simulink model "mc_pos"  (R2021a)
settings: Solver=FixedStepAuto  StartTime=0.0  StopTime=10.0  FixedStep=0.1  RelTol=1e-3
undefined symbols (not defined in the file): CONSTANTS_ONE_G, DiscIntNeverNeededParam, MPC_LAND_SPEED, MPC_SPOOLUP_TIME, MPC_THR_HOVER, MPC_THR_MAX, MPC_THR_MIN, MPC_TILTMAX_AIR, MPC_TILTMAX_LND, MPC_TKO_RAMP_T, MPC_VELD_LP, MPC_XY_P, MPC_XY_VEL_D_ACC, MPC_XY_VEL_I_ACC, MPC_XY_VEL_MAX, MPC_XY_VEL_P_ACC, MPC_Z_P, MPC_Z_VEL_D_ACC, MPC_Z_VEL_I_ACC, MPC_Z_VEL_MAX_DN, MPC_Z_VEL_MAX_UP, MPC_Z_VEL_P_ACC, PX4_TAKEOFF_STATUS, WV_EN
libraries: simulink x16, vrlib x2, sharedtransform x2, aerolibconvert2 x1
(part 3 of 3)

== stateflow chart mc_pos/Flight Mode Manager/Flight Task ==
  state switch_flight_task [parallel]
    en,du:
    start_flight_task();
    handleCommand();
    settings: executionOrder=1
    state Switch_Flight_Task
      state VTOL
        state VTOL_FW_Mode
          en:
          sprintf("Do not run any flight task for VTOLs in fixed-wing mode")
          du:
        state TRANSITION
          en,du:
          task_ == PX4_FLIGHT_TASK.TRANSITION;
        (junction 861) -> VTOL_FW_Mode [order 1] : [vehicle_status.vehicle_type == ...
            | PX4_VEHICLE_STATUS.VEHICLE_TYPE_FIXED_WING]
        (junction 861) -> (junction 859) [order 2]
        (junction 859) -> TRANSITION [order 1] : [vehicle_status.in_transition_mode && ...
            | control_mode.flag_control_altitude_enabled]
      state AUTO
        state AUTO_FOLLOW_ME
          en,du:
          task_ == PX4_FLIGHT_TASK.AUTO_FOLLOW_ME;
        state DESCEND
          en,du:
          task_ == PX4_FLIGHT_TASK.DESCEND;
        state AUTO_LINE_SMOOTH_VEL
          en,du:
          task_ == PX4_FLIGHT_TASK.AUTO_LINE_SMOOTH_VEL;
        (junction 863) -> AUTO_FOLLOW_ME [order 1] : [vehicle_status.nav_state == ...
            | PX4_VEHICLE_STATUS.NAVIGATION_STATE_AUTO_FOLLOW_TARGET]
        (junction 867) -> DESCEND [order 1] : [vehicle_status.nav_state == ...
            | PX4_VEHICLE_STATUS.NAVIGATION_STATE_DESCEND]
        (junction 863) -> (junction 865) [order 2]
        (junction 865) -> (junction 867) [order 2]
        (junction 865) -> AUTO_LINE_SMOOTH_VEL [order 1] : [control_mode.flag_control_auto_enabled]
      state MANUAL
        state MANUAL_POSITION_SMOOTH_VEL
          en,du:
          task_ == PX4_FLIGHT_TASK.MANUAL_POSITION_SMOOTH_VEL;
        state MANUAL_ALTITUDE
          en,du:
          task_ == PX4_FLIGHT_TASK.MANUAL_ALTITUDE;
        state MANUAL_POSITION
          en,du:
          task_ == PX4_FLIGHT_TASK.MANUAL_POSITION;
        state MANUAL_ACCELERATION
          en,du:
          task_ == PX4_FLIGHT_TASK.MANUAL_ACCELERATION;
        state MANUAL_ALTITUDE_SMOOTH_VEL
          en,du:
          task_ == PX4_FLIGHT_TASK.MANUAL_ALTITUDE_SMOOTH_VEL;
        (junction 888) -> MANUAL_POSITION_SMOOTH_VEL [order 1] : [vehicle_status.nav_state == ...
            | PX4_VEHICLE_STATUS.NAVIGATION_STATE_ALTCTL && ...
            | MPC_POS_MODE == 3]
        (junction 872) -> MANUAL_ALTITUDE [order 1] : [vehicle_status.nav_state == ...
            | PX4_VEHICLE_STATUS.NAVIGATION_STATE_ALTCTL && ...
            | MPC_POS_MODE == 0]
        (junction 876) -> (junction 888) [order 2]
        (junction 888) -> (junction 874) [order 2]
        (junction 874) -> (junction 872) [order 2]
        (junction 872) -> (junction 803) [order 2]
        (junction 876) -> MANUAL_POSITION [order 1] : [vehicle_status.nav_state == ...
            | PX4_VEHICLE_STATUS.NAVIGATION_STATE_POSCTL && ...
            | MPC_POS_MODE == 0]
        (junction 874) -> MANUAL_ACCELERATION [order 1] : [vehicle_status.nav_state == ...
            | PX4_VEHICLE_STATUS.NAVIGATION_STATE_POSCTL]
        (junction 803) -> MANUAL_ALTITUDE_SMOOTH_VEL [order 1] : [vehicle_status.nav_state == ....
            | PX4_VEHICLE_STATUS.NAVIGATION_STATE_POSCTL && ...
            | MPC_POS_MODE == 3]
      state OTHER
        state NAVIGATION_STATE_ORBIT
        state None
        (junction 899) -> NAVIGATION_STATE_ORBIT [order 1] : [vehicle_status.nav_state == ...
            | PX4_VEHICLE_STATUS.NAVIGATION_STATE_ORBIT]
        (junction 899) -> None [order 2]
      (default) -> (junction 797)
      (junction 797) -> (junction 861)
      (junction 859) -> (junction 863) [order 2]
      (junction 867) -> (junction 876) [order 2]
      Switch_Flight_Task -> (junction 797) : [hasChanged(local_position.timestamp)]
      (junction 803) -> (junction 899) [order 2]
  state mode_action [parallel]
    settings: executionOrder=2
    state Transition [parallel]
      settings: executionOrder=1
      state running
        en,du:
        % update_initial阶段, 初始化时间和输入数据
        mode_action.FlightTask_updateInitialize();
        % update垂起的过渡阶段，将垂直速度和水平姿态的setpoint点置0
        checkEkfResetCounters();
        acceleration_setpoint(1) = single(0.0);
        acceleration_setpoint(2) = single(0.0);
        position_setpoint = [single(nan); single(nan); single(nan)];
        velocity_setpoint(3) = single(0.0);
        yaw_setpoint = single(nan);
        % update_finalize阶段：在update()之后调用
        %来约束生成的设定值，以符合当前模式的约束
        % update_finalize_none
        takeoff_reactivate
      state not_run
      (default) -> mode_action.Transition.not_run
      mode_action.Transition.not_run -> mode_action.Transition.running : [task_ == PX4_FLIGHT_TASK.TRANSITION]
      mode_action.Transition.running -> mode_action.Transition.not_run : [task_ ~= PX4_FLIGHT_TASK.TRANSITION]
    state AutoFollowMe [parallel]
      settings: executionOrder=2
    state AutoLineSmoothVel [parallel]
      settings: executionOrder=10
      state running
        en,du:
        ext_yaw_handler = weather_vane;
        FlightTaskAuto_updateInitialize
        FlightTaskAutoMapper_update
        FlightTaskAuto_updateFinalize
        takeoff_reactivate
      state not_run
      (default) -> mode_action.AutoLineSmoothVel.not_run
      mode_action.AutoLineSmoothVel.not_run -> mode_action.AutoLineSmoothVel.running : [task_ == PX4_FLIGHT_TASK.AUTO_LINE_SMOOTH_VEL]
      mode_action.AutoLineSmoothVel.running -> mode_action.AutoLineSmoothVel.not_run : [task_ ~= PX4_FLIGHT_TASK.AUTO_LINE_SMOOTH_VEL]
    state Descend [parallel]
      settings: executionOrder=3
    state ManualPosition [parallel]
      settings: executionOrder=4
      state running
        en,du:
        weathervane_yaw_handler = weather_vane;
        % update_initial
        FlightTask_updateInitialize
        Sticks_checkAndSetStickInputs
        % update
        ManualPosition_checkEkfResetCounters
        FlightTaskManualAltitude_updateConstraintsFromEstimator
        ManualPosition_scaleSticks
        ManualPosition_updateSetpoints
        constraints.want_takeoff = (stick_positions_(3) < -0.3);
        % update_final_none
        takeoff_reactivate
      state not_run
      (default) -> mode_action.ManualPosition.not_run
      mode_action.ManualPosition.not_run -> mode_action.ManualPosition.running : [task_==PX4_FLIGHT_TASK.MANUAL_POSITION]
      mode_action.ManualPosition.running -> mode_action.ManualPosition.not_run : [task_~=PX4_FLIGHT_TASK.MANUAL_POSITION]
    state ManualPositionSmoothVel_checking [parallel]
      settings: executionOrder=5
      state not_run
      state running
        en,du:
        weathervane_yaw_handler = weather_vane;
        % update_initial
        mode_action.FlightTask_updateInitialize();
        mode_action.Sticks_checkAndSetStickInputs();
        % update
        ManualPositionSmoothVel_checkEkfResetCounters();
        FlightTaskManualAltitude_updateConstraintsFromEstimator();
        ManualPositionSmoothVel_scaleSticks();
        ManualPositionSmoothVel_updateSetpoints();
        constraints.want_takeoff = (stick_positions_(3) < -0.3);
        % update_finalize_none
        takeoff_reactivate();
      (default) -> mode_action.ManualPositionSmoothVel_checking.not_run
      mode_action.ManualPositionSmoothVel_checking.not_run -> mode_action.ManualPositionSmoothVel_checking.running : [(task_ == PX4_FLIGHT_TASK.MANUAL_POSITION_SMOOTH_VEL)  && ...
          |  (switchTask() == PX4_FLIGHT_TASK_ERROR.NO_ERROR)]
      mode_action.ManualPositionSmoothVel_checking.running -> mode_action.ManualPositionSmoothVel_checking.not_run : [task_ ~= PX4_FLIGHT_TASK.MANUAL_POSITION_SMOOTH_VEL]
    state ManualAcceleration [parallel]
      settings: executionOrder=6
    state ManualAltitude [parallel]
      settings: executionOrder=7
      state running
        en,du:
        % update_initial
        FlightTask_updateInitialize
        Sticks_checkAndSetStickInputs
        % update
        ManualAltitude_checkEkfResetCounters
        FlightTaskManualAltitude_updateConstraintsFromEstimator
        ManualAltitude_scaleSticks
        ManualAltitude_updateSetpoints
        constraints.want_takeoff = (stick_positions_(3) < -0.3);
        % update_finalize_none
        takeoff_reactivate
      state not_run
      (default) -> mode_action.ManualAltitude.not_run
      mode_action.ManualAltitude.not_run -> mode_action.ManualAltitude.running : [task_ == PX4_FLIGHT_TASK.MANUAL_ALTITUDE]
      mode_action.ManualAltitude.running -> mode_action.ManualAltitude.not_run : [task_ ~= PX4_FLIGHT_TASK.MANUAL_ALTITUDE]
    state ManualAltitudeSmoothVel [parallel]
      settings: executionOrder=8
      state running
        en,du:
        % update_initial
        FlightTask_updateInitialize();
        Sticks_checkAndSetStickInputs();
        % update
        ManualAltitudeSmoothVel_checkEkfResetCounters();
        FlightTaskManualAltitude_updateConstraintsFromEstimator();
        ManualAltitudeSmoothVel_scaleSticks();
        ManualAltitudeSmoothVel_updateSetpoints();
        constraints.want_takeoff = (stick_positions_(3) < -0.3);
        % update_finalize_none
        takeoff_reactivate();
      state not_run
      (default) -> mode_action.ManualAltitudeSmoothVel.not_run
      mode_action.ManualAltitudeSmoothVel.not_run -> mode_action.ManualAltitudeSmoothVel.running : [task_==PX4_FLIGHT_TASK.MANUAL_ALTITUDE_SMOOTH_VEL]
      mode_action.ManualAltitudeSmoothVel.running -> mode_action.ManualAltitudeSmoothVel.not_run : [task_~=PX4_FLIGHT_TASK.MANUAL_ALTITUDE_SMOOTH_VEL]
    state Failsafe [parallel]
      settings: executionOrder=9
      state running
        en,du:
        % update initial
        FlightTask_updateInitialize
        % update
        Failsafe_update
        % update_finalize_none
        takeoff_reactivate
      state not_run
      (default) -> mode_action.Failsafe.not_run
      mode_action.Failsafe.not_run -> mode_action.Failsafe.running : [task_ == PX4_FLIGHT_TASK.FAILSAFE]
      mode_action.Failsafe.running -> mode_action.Failsafe.not_run : [task_ ~= PX4_FLIGHT_TASK.FAILSAFE]
  data: out function_output; out function_output; out function_output; out function_output; type local uint8; target_acceptance_radius local single size=1; target local single size=3 =[single(nan); single(nan); single(nan)]; prev_wp local single size=3 =[single(nan); single(nan); single(nan)]; next_wp local single size=3 =[single(nan); single(nan); single(nan)]; mc_cruise_speed local single size=1; reference_position local Bus: px4_reference_position; reference_altitude local single size=1; current_state local Enum: PX4_FLIGHT_TASK_INTERNAL_STATE size=1; closest_pt local single size=2 =[single(nan); single(nan)]; yaw_lock local boolean size=1; wantTakeoff local boolean =false; yaw_sp_aligned local boolean =false; yaw_sp_prev local single size=1 =single(nan); ext_yaw_handler local Bus: px4_weather_vane; trajectory local Bus: px4_mc_pos_traj size=3; out function_output; velocity_scale local single size=1; weathervane_yaw_handler local Bus: px4_weather_vane; result function_output; position_estimate local single size=3; position_lock_active_xy local boolean size=1; position_lock_active_z local boolean size=1; position_setpoint_locked local single size=3; velocity_scale local single size=1; weathervane_yaw_handler local Bus: px4_weather_vane; trajectory local Bus: px4_mc_pos_traj size=3; result function_output; out function_output; position_lock_active_z local boolean size=1; position_setpoint_locked local single size=1; position_estimate local single size=1; trajectory local Bus: px4_mc_pos_traj size=1; out function_output; input_available function_output; dt function_input; time_stretch function_input; traj function_input; out function_output; vel_setpoint function_input; traj function_input; out function_output; traj function_input; n_traj function_input; out function_output; u function_input; out function_output; apply_brake function_input; stopped function_input; d_to_g_lock function_input; out function_output; dcm_z function_input; yyaw function_input; out function_output; weather_vane input Bus: px4_weather_vane size=1; position_setpoint_input input Bus: px4_vehicle_local_position_setpoint; control_mode input Bus: px4_vehicle_control_mode; constraints output Bus: px4_vehicle_constraints; position_ local single size=3; velocity_ local single size=3; yaw_ local single size=1; MPC_XY_CRUISE parameter single; MPC_ACC_HOR parameter single; MPC_JERK_AUTO parameter single; MPC_ACC_DOWN_MAX parameter single; MPC_Z_VEL_MAX_DN parameter single; MPC_XY_VEL_MAX parameter single; dist_to_bottom_ local single size=1; local_position input Bus: px4_vehicle_local_position; home_position input Bus: px4_home_position; dist_to_ground_ local single size=1; triplet_setpoint input Bus: px4_position_setpoint_triplet; MPC_Z_VEL_MAX_UP parameter single; CONSTANTS_RADIUS_OF_EARTH parameter double; MPC_YAW_MODE parameter int32; MPC_ACC_UP_MAX parameter single; MPC_LAND_ALT1 parameter single; MPC_TKO_SPEED parameter single; MPC_TKO_RAMP_T parameter single; manual_control_setpoint input Bus: px4_manual_control_setpoint; positions_expo_ local single size=4 =single([0.0; 0.0; 0.0; 0.0]); vehicle_status input Bus: px4_vehicle_status; MPC_LAND_ALT2 parameter single; MPC_LAND_SPEED parameter single; MPC_LAND_RC_HELP parameter int32; MPC_XY_MAN_EXPO parameter single; MPC_Z_MAN_EXPO parameter single; MPC_YAW_EXPO parameter single; MPC_HOLD_DZ parameter single; NAV_MC_ALT_RAD parameter single; MPC_XY_TRAJ_P parameter single; MPC_XY_ERR_MAX parameter single; deltatime_ local size=1; MPC_YAWRAUTO_MAX parameter single; MIS_YAW_ERR parameter single; MPC_VEL_MANUAL parameter single; stick_positions_ local single size=4 =single([0.0; 0.0; 0.0; 0.0]); MPC_MAN_Y_MAX parameter single; MPC_MAN_Y_TAU parameter single; MPC_JERK_MAX parameter single; MPC_ACC_HOR_MAX parameter single; velocity_setpoint_feedback_ local single size=3; MC_MAN_TILT_TAU parameter single; MPC_MAN_TILT_MAX parameter single; MPC_HOLD_MAX_Z parameter single; MPC_ALT_MODE parameter int32; MPC_HOLD_MAX_XY parameter single; MPC_Z_P parameter single; max_distance_to_ground_ local single size=1; min_distance_to_ground_ local single size=1; max_speed_up_ local single size=1; max_speed_down_ local single size=1; CONSTANTS_ONE_G parameter single size=1; reset_counter_xy_ local uint8 size=1 =uint8(0); reset_counter_vxy_ local uint8 size=1 =uint8(0); reset_counter_z_ local uint8 size=1 =uint8(0); reset_counter_vz_ local uint8 size=1 =uint8(0); reset_counter_heading_ local uint8 size=1 =uint8(0); time_stamp_last_ local size=1 =0; WV_ROLL_MIN parameter single size=1; WV_GAIN parameter single size=1; WV_YRATE_MAX parameter single size=1; WV_EN parameter boolean size=1; task_ local Enum: PX4_FLIGHT_TASK size=1; task_last_ local Enum: PX4_FLIGHT_TASK size=1; MPC_POS_MODE parameter int32 size=1; position_setpoint output single size=3 =[single(nan);single(nan);single(nan)]; velocity_setpoint output single size=3 =[single(nan);single(nan);single(nan)]; acceleration_setpoint output single size=3 =[single(nan);single(nan);single(nan)]; jerk_setpoint output single size=3 =[single(nan);single(nan);single(nan)]; yaw_setpoint output single size=1 =single(nan); yawspeed_setpoint output single size=1 =single(nan); takeoff_state input uint8 size=1; vehicle_command input Bus: px4_vehicle_command size=1
  function start_flight_task:
    | function start_flight_task()
    | 
    | task_failure = false;
    | success = false;
    | task_ = PX4_FLIGHT_TASK.NONE;
    | 
    | % 对于垂起机型处于固定翼模式的时候，拒绝任何flight task
    | if (vehicle_status.vehicle_type == PX4_VEHICLE_STATUS.VEHICLE_TYPE_FIXED_WING)
    |     task_ = PX4_FLIGHT_TASK.NONE;
    |     return
    | end
    | 
    | % 只要在使能高度控制的情况下，才会运行transition flight task（如：高度/位置/自动飞行模式）
    | if (vehicle_status.in_transition_mode && control_mode.flag_control_altitude_enabled)
    |     
    |     task_ = PX4_FLIGHT_TASK.TRANSITION;
    |     
    |     if mode_action.Transition.switchTask
    |         task_last_ = task_;
    |     else
    |         task_ = PX4_FLIGHT_TASK.NONE;
    |     end
    |     
    |     return
    |     
    | end
    | 
    | % 自动跟随模式
    | if (vehicle_status.nav_state == PX4_VEHICLE_STATUS.NAVIGATION_STATE_AUTO_FOLLOW_TARGET)
    |     
    | %     % 暂未实现
    | %     task_ = PX4_FLIGHT_TASK.AUTO_FOLLOW_ME;
    | %     
    | %     if Mode_Action.AutoFollowMe.switchTask
    | %         task_last_ = task_;
    | %     else
    | %         task_failure = true;
    | %     end
    |     
    | elseif (control_mode.flag_control_auto_enabled)
    |     
    |     % AutoLineSmoothVel
    |     task_ = PX4_FLIGHT_TASK.AUTO_LINE_SMOOTH_VEL;
    |     
    |     if mode_action.AutoLineSmoothVel.switchTask
    |         task_last_ = task_;
    |     else
    |         task_failure = true;
    |     end
    |     
    | elseif (vehicle_status.nav_state == PX4_VEHICLE_STATUS.NAVIGATION_STATE_DESCEND)
    |     
    | %     % 紧急降落（暂未实现）
    | %     task_ = PX4_FLIGHT_TASK.DESCEND;
    | %     
    | %     if TASK.Descend.switchTask
    | %         task_last_ = task_;
    | %     else
    | %         task_failure = true;
    | %     end
    | 
    | end
    | 
    | % 手动位置控制模式
    | if (vehicle_status.nav_state == PX4_VEHICLE_STATUS.NAVIGATION_STATE_POSCTL || task_failure)
    |     
    |     switch MPC_POS_MODE
    |         case 0
    |             task_ = PX4_FLIGHT_TASK.MANUAL_POSITION;
    |             success = mode_action.ManualPosition.switchTask;
    |         case 3
    |             task_ = PX4_FLIGHT_TASK.MANUAL_POSITION_SMOOTH_VEL;
    |             success = mode_action.ManualPositionSmoothVel_checking.switchTask;
    |         otherwise
    |             % task_ = PX4_FLIGHT_TASK.MANUAL_ACCELERATION;
    |             % success = TASK.ManualAcceleration.switchTask;
    |     end
    |     
    |     if success
    |         task_last_ = task_;
    |         task_failure = false;
    |     else
    |         task_failure = true;
    |     end
    |     
    | end
    | 
    | % 手动高度控制模式
    | if (vehicle_status.nav_state == PX4_VEHICLE_STATUS.NAVIGATION_STATE_ALTCTL || task_failure)
    |     
    |     switch MPC_POS_MODE
    |         case 0
    |             task_ = PX4_FLIGHT_TASK.MANUAL_ALTITUDE;
    |             success = mode_action.ManualAltitude.switchTask;
    |         case 3
    |             task_ = PX4_FLIGHT_TASK.MANUAL_ALTITUDE_SMOOTH_VEL;
    |             success = mode_action.ManualAltitudeSmoothVel.switchTask;
    |         otherwise
    |             task_ = PX4_FLIGHT_TASK.MANUAL_ALTITUDE_SMOOTH_VEL;
    |             success = mode_action.ManualAltitudeSmoothVel.switchTask;
    |     end
    |     
    |     if success
    |         task_last_ = task_;
    |         task_failure = false;
    |     else
    |         task_failure = true;
    |     end
    |     
    | end
    | 
    | % 检查任务切换是否失败
    | if (task_failure)
    |     
    |     % 由于一些原因导致飞行任务不能启动，这时候进入失效保护模式
    |     task_ = PX4_FLIGHT_TASK.FAILSAFE;
    |     
    |     if mode_action.Failsafe.switchTask
    |         task_last_ = task_;
    |     else
    |         task_ = PX4_FLIGHT_TASK.NONE;
    |     end
    |     
    | end
    | 
    | end
  function handleCommand:
    | function handleCommand()
    | 
    | % 如果vehicle_command主题有更新
    | if (hasChanged(vehicle_command.timestamp))
    |     % 暂未实现功能：
    |     % 1.判断是否成功切换到的期望的任务（desired task）,主要是处理“刷锅”模式的，判断中心坐标和刷锅高度是否正确;
    |     % 2.发布command_ack;
    | end
    | 
    | end
  function checkEkfResetCounters:
    | function checkEkfResetCounters()
    | 
    | if (local_position.xy_reset_counter ~= reset_counter_xy_)
    |     reset_counter_xy_ = local_position.xy_reset_counter;
    | end
    | 
    | if (local_position.vxy_reset_counter ~= reset_counter_vxy_)
    |     reset_counter_vxy_ = local_position.vxy_reset_counter;
    | end
    | 
    | if (local_position.z_reset_counter ~= reset_counter_z_)
    |     reset_counter_z_ = local_position.z_reset_counter;
    | end
    | 
    | if (local_position.vz_reset_counter ~= reset_counter_vz_)
    |     reset_counter_vz_ = local_position.vz_reset_counter;
    | end
    | 
    | if (local_position.heading_reset_counter ~= reset_counter_heading_)
    |     reset_counter_heading_ = local_position.heading_reset_counter;
    | end
    | 
    | end
  function takeoff_reactivate:
    | function takeoff_reactivate
    | 
    | if (takeoff_state < uint8(PX4_TAKEOFF_STATUS.TAKEOFF_STATE_RAMPUP))
    |     FlightTask_activate;
    | end
    | 
    | end
  function out = switchTask:
    | function out = switchTask
    | out = true;
    | 
    | if task_ ~= task_last_
    |     FlightTask_updateInitialize;
    |     FlightTask_activate;
    | end
    | 
    | end
  function checkEkfResetCounters:
    | function checkEkfResetCounters
    | 
    | if local_position.xy_reset_counter ~= reset_counter_xy_
    |     reset_counter_xy_ = local_position.xy_reset_counter;
    |     
    |     trajectory(1).state_x = position_(1);
    |     trajectory(1).state_init_x = position_(1);
    |     trajectory(2).state_x = position_(2);
    |     trajectory(2).state_init_x = position_(2);
    | end
    | 
    | if local_position.vxy_reset_counter ~= reset_counter_vxy_
    |     reset_counter_vxy_ = local_position.vxy_reset_counter;
    |     
    |     trajectory(1).state_v = velocity_(1);
    |     trajectory(1).state_init_v = velocity_(1);
    |     trajectory(2).state_v = velocity_(2);
    |     trajectory(2).state_init_v = velocity_(2);
    | end
    | 
    | if local_position.z_reset_counter ~= reset_counter_z_
    |     reset_counter_z_ = local_position.z_reset_counter;
    |     
    |     trajectory(3).state_x = position_(3);
    |     trajectory(3).state_init_x = position_(3);
    | end
    | 
    | if local_position.vz_reset_counter ~= reset_counter_vz_
    |     reset_counter_vz_ = local_position.vz_reset_counter;
    |     
    |     trajectory(3).state_v = velocity_(3);
    |     trajectory(3).state_init_v = velocity_(3);
    | end
    | 
    | if local_position.heading_reset_counter ~= reset_counter_heading_
    |     reset_counter_heading_ = local_position.heading_reset_counter;
    |     
    |     yaw_sp_prev = yaw_sp_prev + local_position.delta_heading;
    | end
    | 
    | end
  function FlightTaskAutoMapper_update:
    | function FlightTaskAutoMapper_update
    | persistent type_previous
    | if isempty(type_previous)
    |     type_previous = uint8(PX4_POSITION_SETPOINT.SETPOINT_TYPE_IDLE);
    | end
    | 
    | %% 
    | checkEkfResetCounters;
    | 
    | %% setConstraints
    | constraints.speed_xy = min(MPC_XY_VEL_MAX, MPC_XY_CRUISE);
    | constraints.speed_up = single(MPC_Z_VEL_MAX_UP);
    | constraints.speed_down = single(MPC_Z_VEL_MAX_DN);
    | constraints.want_takeoff = false;
    | 
    | %% prepare_setpoint
    | if type_previous == uint8(PX4_POSITION_SETPOINT.SETPOINT_TYPE_IDLE)
    |     acceleration_setpoint = [single(nan); single(nan); single(nan)];
    | end
    | 
    | switch type
    |     case uint8(PX4_POSITION_SETPOINT.SETPOINT_TYPE_IDLE)
    |         position_setpoint = [single(nan); single(nan); single(nan)];
    |         velocity_setpoint = [single(nan); single(nan); single(nan)];
    |         acceleration_setpoint = [single(0); single(0); single(100)];
    |         
    |     case uint8(PX4_POSITION_SETPOINT.SETPOINT_TYPE_LAND)
    |         position_setpoint = [target(1); target(2); single(nan)];
    |         velocity_setpoint = [single(nan); single(nan); getLandSpeed];
    |         
    |     case {uint8(PX4_POSITION_SETPOINT.SETPOINT_TYPE_LOITER),uint8(PX4_POSITION_SETPOINT.SETPOINT_TYPE_POSITION)}
    |         position_setpoint = target;
    |         velocity_setpoint = [single(nan); single(nan); single(nan)];
    |         
    |     case uint8(PX4_POSITION_SETPOINT.SETPOINT_TYPE_TAKEOFF)
    |         position_setpoint = target;
    |         velocity_setpoint = [single(nan); single(nan); single(nan)];
    |         
    |     case uint8(PX4_POSITION_SETPOINT.SETPOINT_TYPE_VELOCITY)
    |         position_setpoint = [single(nan); single(nan); position_(3)];
    |         vel_sp_xy = vector2_unit_or_zero([velocity_(1), velocity_(2)]);
    |         velocity_setpoint = [mc_cruise_speed * vel_sp_xy(1); mc_cruise_speed * vel_sp_xy(2); single(nan)];
    |         
    |     otherwise
    |         position_setpoint = target;
    |         velocity_setpoint = [single(nan); single(nan); single(nan)];
    | end
    | 
    | %% 
    | generateSetpoints
    | type_previous = type;
    | 
    | end
    | 
    | %% 
    | function y = getLandSpeed
    | 
    | y = gradual(dist_to_ground_, MPC_LAND_ALT2, MPC_LAND_ALT1, MPC_LAND_SPEED, constraints.speed_down);
    | 
    | if MPC_LAND_RC_HELP && (dist_to_ground_ < MPC_LAND_ALT1) && Sticks_checkAndSetStickInputs
    |     y = y * (1 + positions_expo_(3));
    | end
    | 
    | end
  function generateSetpoints:
    | function generateSetpoints
    | 
    | persistent max_speed_prev
    | if isempty(max_speed_prev)
    |     max_speed_prev = single(0);
    | end
    | 
    | jerk_sp_smooth = [single(nan); single(nan); single(nan)];
    | accel_sp_smooth = [single(nan); single(nan); single(nan)];
    | vel_sp_smooth = [single(nan); single(nan); single(nan)];
    | pos_sp_smooth = [single(nan); single(nan); single(nan)];
    | 
    | %% updateTurningCheck
    | vel_traj = [trajectory(1).state_v, trajectory(2).state_v];
    | pos_trajj = [trajectory(1).state_x, trajectory(2).state_x];
    | target_xy = [target(1), target(2)];
    | u_vel_traj = vector2_unit_or_zero(vel_traj);
    | pos_to_target = target_xy - pos_trajj;
    | cos_align = dot(u_vel_traj, vector2_unit_or_zero(pos_to_target));
    | 
    | is_turning = (norm(vel_traj)^2 > 0.2^2) && cos_align < 0.98 && (norm(pos_to_target)^2 > target_acceptance_radius^2);
    | 
    | %% prepareSetpoints
    | wantTakeoff = false;
    | 
    | if (MPC_YAW_MODE == 4) && ~yaw_sp_aligned
    |     velocity_setpoint = [single(0); single(0); single(0)];
    |     
    | else
    |     xy_pos_setpoint_valid = isfinite(position_setpoint(1)) && isfinite(position_setpoint(2));
    |     z_pos_setpoint_valid = isfinite(position_setpoint(3));
    |     
    |     if xy_pos_setpoint_valid && z_pos_setpoint_valid
    |         pos_traj = [trajectory(1).state_x; trajectory(2).state_x; trajectory(3).state_x];
    |         u_pos_traj_to_dest = vector3_unit_or_zero(getCrossingPoint(is_turning) - pos_traj);
    |         
    |         xy_speed = getMaxXYSpeed;
    |         z_speed = getMaxZSpeed;
    |         
    |         if is_turning
    |             xy_speed = min(max_speed_prev, xy_speed);
    |         else
    |             max_speed_prev = xy_speed;
    |         end
    |         
    |         vel_sp_constrained = u_pos_traj_to_dest * sqrt(xy_speed^2 + z_speed^2);
    |         vel_sp_constrained = clampToXYNorm(vel_sp_constrained, xy_speed, 0.5);
    |         vel_sp_constrained = clampToZNorm(vel_sp_constrained, z_speed, 0.5);
    |         
    |         for i = 1:1:3
    |             if isfinite(velocity_setpoint(i))
    |                 velocity_setpoint(i) = velocity_setpoint(i) + vel_sp_constrained(i);
    |             else
    |                 velocity_setpoint(i) = vel_sp_constrained(i);
    |             end
    |         end
    |         
    |     end
    |     
    |     if xy_pos_setpoint_valid && ~z_pos_setpoint_valid
    |         ppos_traj = [trajectory(1).state_x, trajectory(2).state_x];
    |         a = getCrossingPoint(is_turning);
    |         pos_traj_to_dest_xy = [a(1), a(2)] - ppos_traj;
    |         u_pos_traj_to_dest_xy = vector2_unit_or_zero(pos_traj_to_dest_xy);
    |         
    |         xy_speed = getMaxXYSpeed;
    |         
    |         if is_turning
    |             xy_speed = min(max_speed_prev, xy_speed);
    |         else
    |             max_speed_prev = xy_speed;
    |         end
    |         
    |         vel_sp_constrained_xy = u_pos_traj_to_dest_xy * xy_speed;
    |         
    |         for i = 1:1:2
    |             if isfinite(velocity_setpoint(i))
    |                 velocity_setpoint(i) = velocity_setpoint(i) + vel_sp_constrained_xy(i);
    |             else
    |                 velocity_setpoint(i) = vel_sp_constrained_xy(i);
    |             end
    |         end
    |     end
    |     
    |     if ~xy_pos_setpoint_valid && z_pos_setpoint_valid
    |         z_dir = sign(position_setpoint(3) - trajectory(3).state_x);
    |         vel_sp_z = z_dir * getMaxZSpeed;
    |         
    |         if isfinite(velocity_setpoint(3))
    |             velocity_setpoint(2) = velocity_setpoint(2) + vel_sp_z;
    |         else
    |             velocity_setpoint(2) = vel_sp_z;
    |         end
    |         
    |     end
    |     
    |     wantTakeoff = (velocity_setpoint(3) < -0.3);
    | end
    | 
    | %% generateTrajectory
    | position_trajectory_xy = [trajectory(1).state_x, trajectory(2).state_x];
    | position_xy = [position_(1), position_(2)];
    | vel_traj_xy = [trajectory(1).state_v, trajectory(2).state_v];
    | drone_to_trajectory_xy = position_trajectory_xy - position_xy;
    | position_error = norm(drone_to_trajectory_xy);
    | 
    | time_stretch = 1 - constrain(position_error / MPC_XY_ERR_MAX, 0, 1);
    | if dot(drone_to_trajectory_xy, vel_traj_xy) < single(0)
    |     time_stretch = single(1);
    | end
    | 
    | for i = 1:1:3
    |     trajectory(i) = VelocitySmoothing_updateTraj(deltatime_,time_stretch,trajectory(i));
    |     jerk_sp_smooth(i) = trajectory(i).state_j;
    |     accel_sp_smooth(i) = trajectory(i).state_a;
    |     vel_sp_smooth(i) = trajectory(i).state_v;
    |     pos_sp_smooth(i) = trajectory(i).state_x;
    | end
    | 
    | updateTrajConstraints;
    | 
    | for i = 1:1:3
    |     trajectory(i) = VelocitySmoothing_updateDurations(velocity_setpoint(i),trajectory(i));
    | end
    | % Synchronize XYZ trajectories to have the same total time. This is required to generate straight lines.
    | trajectory = VelocitySmoothing_timeSynchronization(trajectory, 3);
    | 
    | %% output
    | jerk_setpoint = jerk_sp_smooth;
    | acceleration_setpoint = accel_sp_smooth;
    | velocity_setpoint = vel_sp_smooth;
    | position_setpoint = pos_sp_smooth;
    | 
    | if ~isfinite(yaw_setpoint) && ~isfinite(yawspeed_setpoint)
    |     generateHeading;
    | end
    | 
    | end
    | 
    | %% 
    | function y = getCrossingPoint(turning)
    | 
    | y = position_setpoint;
    | 
    | if ~isTargetModified
    |     if turning
    |         a = getL1Point;
    |         y(1) = a(1);
    |         y(2) = a(2);
    |         y(3) = target(3);
    |     else
    |         y = target;
    |     end
    | end
    | 
    | end
    | 
    | %% 
    | function y = getMaxXYSpeed
    | 
    | pos_traj = [trajectory(1).state_x; trajectory(2).state_x; trajectory(3).state_x];
    | config_z_accept_rad = NAV_MC_ALT_RAD;
    | config_xy_accept_rad = target_acceptance_radius;
    | config_max_acc_xy = trajectory(1).max_accel;
    | config_max_jerk = trajectory(1).max_jerk;
    | config_max_speed_xy = mc_cruise_speed;
    | config_max_acc_xy_radius_scale = MPC_XY_TRAJ_P;
    | 
    | waypoints = [pos_traj, target, next_wp];
    | 
    | if isTargetModified
    |     waypoints = [pos_traj, position_setpoint, position_setpoint];
    | end
    | 
    | y = computeXYSpeedFromWaypoints(waypoints, config_z_accept_rad, config_xy_accept_rad, config_max_acc_xy, config_max_jerk, config_max_speed_xy, config_max_acc_xy_radius_scale);
    | 
    | end
    | 
    | %% 
    | function y = getMaxZSpeed
    | 
    | z_setpoint = target(3);
    | z_modified = isfinite(position_setpoint(3)) && (abs(target(3) - position_setpoint(3)) > eps);
    | 
    | if z_modified
    |     z_setpoint = position_setpoint(3);
    | end
    | 
    | distance_start_target = abs(z_setpoint - trajectory(3).state_x);
    | y = min(trajectory(3).max_vel, computeMaxSpeedFromDistance(trajectory(3).max_jerk, trajectory(3).max_accel, distance_start_target, single(0)));
    | 
    | end
    | 
    | %% 
    | function y = isTargetModified
    | 
    | a = [target(1) - position_setpoint(1), target(2) - position_setpoint(2)];
    | xy_modified = norm(a)^2 > eps^2;
    | z_modified = isfinite(position_setpoint(3)) && (abs(target(3) - position_setpoint(3)) > eps);
    | 
    | y = xy_modified || z_modified;
    | 
    | end
    | 
    | %% 
    | function y = getL1Point
    | 
    | pos_traj = [trajectory(1).state_x, trajectory(2).state_x];
    | target_xy = [target(1), target(2)];
    | u_prev_to_target = vector2_unit_or_zero([target_xy(1) - prev_wp(1), target_xy(2) - prev_wp(2)]);
    | prev_to_pos = [pos_traj(1) - prev_wp(1), pos_traj(2) - prev_wp(2)];
    | prev_to_closest = u_prev_to_target * (dot(prev_to_pos, u_prev_to_target) / norm(u_prev_to_target));
    | closest_pt1 = [prev_wp(1) + prev_to_closest(1), prev_wp(2) + prev_to_closest(2)];
    | 
    | % Compute along-track error using L1 distance and cross-track error
    | crosstrack_error = norm(closest_pt1 - pos_traj);
    | 
    | l1 = max(target_acceptance_radius, single(5));
    | alongtrack_error = single(0);
    | 
    | if l1 > crosstrack_error
    |     alongtrack_error = sqrt(l1^2 - crosstrack_error^2);
    | end
    | 
    | y = closest_pt1 + alongtrack_error * u_prev_to_target;
    | 
    | end
    |  
    | %% 
    | function generateHeading
    | 
    | if ~generateHeadingAlongTraj
    |     yaw_setpoint = yaw_sp_prev;
    | end
    | 
    | end
    | 
    | %% 
    | function y = generateHeadingAlongTraj
    | 
    | y = false;
    | vel_sp_xy = [velocity_setpoint(1), velocity_setpoint(2)];
    | traj_to_target = [target(1) - position_(1), target(2) - position_(2)];
    | 
    | if (norm(vel_sp_xy) > single(0.1)) && (norm(traj_to_target) > single(2))
    |     yaw_setpoint = compute_heading_from_2D_vector(yaw_setpoint, vel_sp_xy);
    |     y = true;
    | end
    | 
    | end
  function FlightTaskAuto_updateFinalize:
    | function FlightTaskAuto_updateFinalize
    | 
    | yawrate_max = deg2rad(MPC_YAWRAUTO_MAX);
    | yaw_sp_aligned = true;
    | 
    | if isfinite(yaw_setpoint) && isfinite(yaw_sp_prev)
    |     dyaw_desired = wrap(yaw_setpoint - yaw_sp_prev, -single(pi), single(pi));
    |     dyaw = constrain(dyaw_desired, -yawrate_max * deltatime_, yawrate_max * deltatime_);
    |     yaw_setpoint_sat = wrap(yaw_sp_prev + dyaw, -single(pi), single(pi));
    |     
    |     yaw_sp_aligned = (abs(wrap(yaw_setpoint - yaw_setpoint_sat, -single(pi), single(pi))) < deg2rad(MIS_YAW_ERR));
    |     
    |     yaw_setpoint = yaw_setpoint_sat;
    |     yaw_sp_prev = yaw_setpoint;
    |     
    |     if ~isfinite(yawspeed_setpoint) && (deltatime_ > eps)
    |         yawspeed_setpoint = dyaw / deltatime_;
    |     end
    | end
    | 
    | if isfinite(yawspeed_setpoint)
    |     yaw_sp_aligned = yaw_sp_aligned && (abs(yawspeed_setpoint) < yawrate_max);
    |     yawspeed_setpoint = constrain(yawspeed_setpoint, -yawrate_max, yawrate_max);
    | end
    | 
    | constraints.want_takeoff = wantTakeoff;
    | 
    | end
  function takeoff_reactivate:
    | function takeoff_reactivate
    | 
    | if takeoff_state < uint8(PX4_TAKEOFF_STATUS.TAKEOFF_STATE_RAMPUP)
    |     FlightTask_activate;
    |     
    |     for i=1:1:3
    |         trajectory(i).state_j = single(0);
    |         trajectory(i).state_a = single(0);
    |         trajectory(i).state_v = single(0);
    |         trajectory(i).state_x = position_(i);
    |         if i==3
    |             trajectory(i).state_v = single(0.7);
    |         end
    |         
    |         trajectory(i).state_init_x = trajectory(i).state_x;
    |         trajectory(i).state_init_v = trajectory(i).state_v;
    |         trajectory(i).state_init_a = trajectory(i).state_a;
    |         trajectory(i).state_init_j = trajectory(i).state_j;
    |     end
    | end
    | 
    | end
  function out = evaluateGlobalReference:
    | function out = evaluateGlobalReference
    | 
    | if local_position.z_global
    |     reference_altitude = local_position.ref_alt;
    | else
    |     reference_altitude = single(0);
    | end
    | 
    | if local_position.xy_global
    |     ref_lat = local_position.ref_lat;
    |     ref_lon = local_position.ref_lon;
    | else
    |     ref_lat = double(0);
    |     ref_lon = double(0);
    | end
    | 
    | reference_position = map_projection_init_timestamped(ref_lat, ref_lon, uint64(0));
    | 
    | out = isfinite(reference_altitude) && isfinite(ref_lat) && isfinite(ref_lon);
    | 
    | end
  function out = switchTask:
    | function out = switchTask
    | out = true;
    | 
    | if task_ ~= task_last_
    |     % getPositionSetpoint
    |     last_setpoint.x = position_setpoint(1);
    |     last_setpoint.y = position_setpoint(2);
    |     last_setpoint.z = position_setpoint(3);
    | 
    |     last_setpoint.vx = velocity_setpoint(1);
    |     last_setpoint.vy = velocity_setpoint(2);
    |     last_setpoint.vz = velocity_setpoint(3);
    | 
    |     last_setpoint.yaw = yaw_setpoint;
    |     last_setpoint.yawspeed = yawspeed_setpoint;
    | 
    |     last_setpoint.acceleration = acceleration_setpoint;
    |     last_setpoint.jerk = jerk_setpoint;
    |     last_setpoint.thrust = [single(nan); single(nan); single(nan)];
    | 
    |     % updateInitialize
    |     flag_init = FlightTaskAuto_updateInitialize;
    | 
    |     % activate
    |     FlightTask_activate;
    | 
    |     position_setpoint = position_;
    |     velocity_setpoint = velocity_;
    |     yaw_setpoint = yaw_;
    |     yawspeed_setpoint = single(0);
    | 
    |     constraints.speed_xy = min(constraints.speed_xy, MPC_XY_CRUISE);
    |     if (~isfinite(last_setpoint.yaw))
    |         last_setpoint.yaw = yaw_;
    |     end
    |     yaw_sp_prev = last_setpoint.yaw
    | 
    |     vel_prev = [last_setpoint.vx, last_setpoint.vy, last_setpoint.vz];
    |     pos_prev = [last_setpoint.x, last_setpoint.y, last_setpoint.z];
    | 
    |     for i=1:1:3
    |         trajectory(i).state_x = IsFinite(pos_prev(i), position_(i));
    |         trajectory(i).state_v = IsFinite(vel_prev(i), velocity_(i));
    |         trajectory(i).state_a = IsFinite(last_setpoint.acceleration(i), single(0));
    |         trajectory(i).state_j = single(0);
    | 
    |         trajectory(i).state_init_x = trajectory(i).state_x;
    |         trajectory(i).state_init_v = trajectory(i).state_v;
    |         trajectory(i).state_init_a = trajectory(i).state_a;
    |         trajectory(i).state_init_j = trajectory(i).state_j;
    |     end
    | 
    |     updateTrajConstraints;
    |     
    |     out = flag_init;
    | %     out = true;
    | end
    | 
    | end
  function evaluateTriplets:
    | function evaluateTriplets()
    | 
    | persistent triplet_target triplet_prev_wp triplet_next_wp lock_position_xy prev_was_valid next_was_valid prev_prev_wp
    | if isempty(triplet_target)
    |     triplet_target = single([nan; nan; nan]);
    | end
    | if isempty(triplet_prev_wp)
    |     triplet_prev_wp = single([nan; nan; nan]);
    | end
    | if isempty(triplet_next_wp)
    |     triplet_next_wp = single([nan; nan; nan]);
    | end
    | if isempty(prev_prev_wp)
    |     prev_prev_wp = single([nan; nan; nan]);
    | end
    | if isempty(lock_position_xy)
    |     lock_position_xy = [single(nan); single(nan)];
    | end
    | if isempty(prev_was_valid)
    |     prev_was_valid = false;
    | end
    | if isempty(next_was_valid)
    |     next_was_valid = false;
    | end
    | 
    | if ~triplet_setpoint.current.valid || ~isfinite(triplet_setpoint.current.alt)
    |     triplet_next_wp = position_;
    |     triplet_target = position_;
    |     triplet_prev_wp = position_;
    |     prev_prev_wp = position_;
    |     type = uint8(PX4_POSITION_SETPOINT.SETPOINT_TYPE_LOITER);
    |     yaw_setpoint = yaw_;
    |     yawspeed_setpoint = single(nan);
    |     target_acceptance_radius = triplet_setpoint.current.acceptance_radius;
    |     
    |     [target, prev_wp, next_wp] = updateInternalWaypoints(triplet_target, triplet_next_wp, triplet_prev_wp);
    |     
    | else
    |     type = triplet_setpoint.current.type;
    |     
    |     mc_cruise_speed = triplet_setpoint.current.cruising_speed;
    |     if ~isfinite(mc_cruise_speed) || (mc_cruise_speed < 0)
    |         mc_cruise_speed = constraints.speed_xy;
    |     end
    |     mc_cruise_speed = min(mc_cruise_speed, MPC_XY_VEL_MAX);
    |     
    |     tmp_target = single([nan; nan; nan]);
    |     
    |     if ~isfinite(triplet_setpoint.current.lat) || ~isfinite(triplet_setpoint.current.lon)
    |         if ~isfinite(lock_position_xy(1))
    |             lock_position_xy(1) = position_(1);
    |             tmp_target(1) = position_(1);
    |             lock_position_xy(2) = position_(2);
    |             tmp_target(2) = position_(2);
    |         else
    |             tmp_target(1) = lock_position_xy(1);
    |             tmp_target(2) = lock_position_xy(2);
    |         end
    |     else
    |         lock_position_xy = [single(nan); single(nan)];
    |         [tmp_target(1), tmp_target(2)] = map_projection_project(reference_position, triplet_setpoint.current.lat, triplet_setpoint.current.lon, CONSTANTS_RADIUS_OF_EARTH);
    |     end
    |     
    |     tmp_target(3) = -(triplet_setpoint.current.alt - reference_altitude);
    |     
    |     triplet_update = true;
    |     prev_next_validity_changed = (prev_was_valid ~= triplet_setpoint.previous.valid) || (next_was_valid ~= triplet_setpoint.next.valid);
    |     
    |     if isfinite(triplet_target(1)) && isfinite(triplet_target(2)) && isfinite(triplet_target(3)) && (abs(triplet_target(1) - tmp_target(1)) < 0.001)...
    |             && (abs(triplet_target(2) - tmp_target(2)) < 0.001) && (abs(triplet_target(3) - tmp_target(3)) < 0.001) && ~prev_next_validity_changed
    |         
    |         triplet_update = false;
    |     else
    |         triplet_target = tmp_target;
    |         target_acceptance_radius = triplet_setpoint.current.acceptance_radius;
    |         
    |         if ~isfinite(triplet_target(1)) || ~isfinite(triplet_target(2))
    |             triplet_target(1) = position_(1);
    |             triplet_target(2) = position_(2);
    |         end
    |         if ~isfinite(triplet_target(3))
    |             triplet_target(3) = position_(3);
    |         end
    |         
    |         prev_prev_wp = triplet_prev_wp;
    |         if isfinite(triplet_setpoint.previous.lat) && isfinite(triplet_setpoint.previous.lon) && isfinite(triplet_setpoint.previous.alt) && triplet_setpoint.previous.valid
    |             [triplet_prev_wp(1), triplet_prev_wp(2)] = map_projection_project(reference_position, triplet_setpoint.previous.lat, triplet_setpoint.previous.lon, CONSTANTS_RADIUS_OF_EARTH);
    |             triplet_prev_wp(3) = -(triplet_setpoint.previous.alt - reference_altitude);
    |         else
    |             triplet_prev_wp = position_;
    |         end
    |         prev_was_valid = triplet_setpoint.previous.valid;
    |         
    |         if isfinite(triplet_setpoint.next.lat) && isfinite(triplet_setpoint.next.lon) && isfinite(triplet_setpoint.next.alt) && triplet_setpoint.next.valid
    |             [triplet_next_wp(1), triplet_next_wp(2)] = map_projection_project(reference_position, triplet_setpoint.next.lat, triplet_setpoint.next.lon, CONSTANTS_RADIUS_OF_EARTH);
    |             triplet_next_wp(3) = -(triplet_setpoint.next.alt - reference_altitude);
    |         else
    |             triplet_next_wp = triplet_target;
    |         end
    |         next_was_valid = triplet_setpoint.next.valid;
    |     end
    |     
    |     if ~isempty(fieldnames(ext_yaw_handler))   % if structure---ext_yaw_handler is null, the return value is 1, or it will be 0
    |         if WV_EN && ~triplet_setpoint.current.disable_weather_vane
    |             ext_yaw_handler.is_active = true;
    |         else
    |             ext_yaw_handler.is_active = false;
    |         end
    |     end
    | 
    |     previous_state = current_state;
    |     current_state = getCurrentState(triplet_target, triplet_prev_wp);
    |     
    |     if triplet_update || (current_state ~= previous_state) || (current_state == PX4_FLIGHT_TASK_INTERNAL_STATE.TARGET_BEHIND)
    |         [target, prev_wp, next_wp] = updateInternalWaypoints(triplet_target, triplet_next_wp, triplet_prev_wp);
    |         yaw_lock = false;
    |     end
    |     
    |     if ~isempty(fieldnames(ext_yaw_handler)) && ext_yaw_handler.is_active   % if structure---ext_yaw_handler is null, the return value is 1, or it will be 0
    |         yaw_setpoint = yaw_;
    |         
    |         if norm([velocity_setpoint(1), velocity_setpoint(2)])^2 > (MPC_XY_CRUISE / 2)^2
    |             yawspeed_setpoint = single(0);
    |         else
    |             yawspeed_setpoint = get_weathervane_yawrate(ext_yaw_handler.dcm_z_sp_prev, ext_yaw_handler.yaw);
    |         end
    |         
    |     elseif (type == uint8(PX4_POSITION_SETPOINT.SETPOINT_TYPE_FOLLOW_TARGET)) && triplet_setpoint.current.yawspeed_valid
    |         yawspeed_setpoint = triplet_setpoint.current.yawspeed;
    |         yaw_setpoint = single(nan);
    |         
    |     else
    |         yawspeed_setpoint = single(nan);
    |         
    |         if ((type ~= uint8(PX4_POSITION_SETPOINT.SETPOINT_TYPE_TAKEOFF)) || triplet_setpoint.current.disable_weather_vane) && triplet_setpoint.current.yaw_valid
    |             yaw_setpoint = triplet_setpoint.current.yaw;
    |             
    |         else
    |             set_heading_from_mode;
    |         end
    |     end
    |     
    | end
    | 
    | end
    | 
    | %% 
    | function [target1, prev1, next1] = updateInternalWaypoints(triplet_target, triplet_next_wp, triplet_prev_wp)
    | 
    | switch current_state
    |     case PX4_FLIGHT_TASK_INTERNAL_STATE.TARGET_BEHIND
    |         target1 = triplet_target;
    |         prev1 = position_;
    |         next1 = triplet_next_wp;
    |         
    |     case PX4_FLIGHT_TASK_INTERNAL_STATE.PREVIOUS_IN_FRONT
    |         next1 = triplet_target;
    |         target1 = triplet_prev_wp;
    |         prev1 = position_;
    |         
    |     case PX4_FLIGHT_TASK_INTERNAL_STATE.TARGET_BEHIND
    |         next1 = triplet_target;
    |         target1 = [closest_pt(1); closest_pt(2); triplet_target(3)];
    |         prev1 = position_;
    |         
    |     otherwise
    |         target1 = triplet_target;
    |         prev1 = triplet_prev_wp;
    |         next1 = triplet_next_wp;
    | end
    | 
    | end
    | 
    | %% 
    | function y = getCurrentState(target1, prev)
    |     u_prev_to_target = vector2_unit_or_zero([target1(1) - prev(1), target1(2) - prev(2)]);
    |     
    |     pos_to_target = [target1(1) - position_(1), target1(2) - position_(2)];
    |     prev_to_pos = [position_(1) - prev(1), position_(2) - prev(2)];
    |     
    |     b = [prev(1), prev(2)] + u_prev_to_target * dot(prev_to_pos, u_prev_to_target);
    |     closest_pt = b';
    |     
    |     if (dot(u_prev_to_target, pos_to_target) / norm(pos_to_target)) < 0
    |         y = PX4_FLIGHT_TASK_INTERNAL_STATE.TARGET_BEHIND;
    |         
    |     elseif (norm(prev_to_pos) > target_acceptance_radius) && ((dot(u_prev_to_target, prev_to_pos) / norm(prev_to_pos)) < 0)
    |         y = PX4_FLIGHT_TASK_INTERNAL_STATE.PREVIOUS_IN_FRONT;
    |         
    |     elseif (norm([position_(1) - closest_pt(1), position_(2) - closest_pt(2)])) > target_acceptance_radius
    |         y = PX4_FLIGHT_TASK_INTERNAL_STATE.TARGET_BEHIND;
    |         
    |     else
    |         y = PX4_FLIGHT_TASK_INTERNAL_STATE.NONE;
    |     end
    | 
    | end
    | 
    | %% 
    | function set_heading_from_mode
    | 
    | v = [single(0), single(0)];
    | 
    | switch MPC_YAW_MODE
    |     case 0
    |     case 4
    |         v = [target(1) - position_(1), target(2) - position_(2)];
    |         
    |     case 1
    |         if home_position.valid_lpos
    |             v = [home_position.x - position_(1), home_position.y - position_(2)];
    |         end
    |         
    |     case 2
    |         if home_position.valid_lpos
    |             v = [position_(1) - home_position.x, position_(2) - home_position.y];
    |         end
    |         
    |     case 3
    |         v = [single(nan), single(nan)];
    |         
    |     otherwise
    |         v = [single(0), single(0)];       
    | end
    | 
    | if isfinite(norm(v))
    |     if ~yaw_lock
    |         
    |         if norm(v) < target_acceptance_radius
    |             yaw_setpoint = yaw_;
    |             yaw_lock = true;
    |         else
    |             yaw_setpoint = compute_heading_from_2D_vector(yaw_setpoint, v);
    |         end
    |         
    |     end
    | else
    |     yaw_lock = false;
    |     yaw_setpoint = single(nan);
    | end
    | 
    | end
  function out = FlightTaskAuto_updateInitialize:
    | function out = FlightTaskAuto_updateInitialize
    | 
    | FlightTask_updateInitialize;
    | out = evaluateGlobalReference;
    | evaluateTriplets;
    | 
    | out = out && isfinite(position_(1)) && isfinite(position_(2)) && isfinite(position_(3)) && isfinite(velocity_(1)) && isfinite(velocity_(2)) && isfinite(velocity_(3));
    | 
    | end
  function updateTrajConstraints:
    | function updateTrajConstraints
    | 
    | trajectory(1).max_accel = single(MPC_ACC_HOR);
    | trajectory(2).max_accel = single(MPC_ACC_HOR);
    | trajectory(1).max_vel = single(MPC_XY_VEL_MAX);
    | trajectory(2).max_vel = single(MPC_XY_VEL_MAX);
    | trajectory(1).max_jerk = single(MPC_JERK_AUTO);
    | trajectory(2).max_jerk = single(MPC_JERK_AUTO);
    | trajectory(3).max_jerk = single(MPC_JERK_AUTO);
    | 
    | if velocity_setpoint(3) < 0   % UP
    |     trajectory(3).max_accel = MPC_ACC_UP_MAX;
    |     trajectory(3).max_vel = MPC_Z_VEL_MAX_UP;
    |     
    |     if (type == uint8(PX4_POSITION_SETPOINT.SETPOINT_TYPE_TAKEOFF)) && (dist_to_ground_ < MPC_LAND_ALT1)
    |         trajectory(3).max_vel = MPC_TKO_SPEED;
    |         trajectory(3).max_accel = min(trajectory(3).max_accel, MPC_TKO_SPEED / MPC_TKO_RAMP_T);
    |         
    |         trajectory(3).state_x = position_(3);
    |         trajectory(3).state_init_x = trajectory(3).state_x;
    |     end
    | else
    |     trajectory(3).max_accel = single(MPC_ACC_DOWN_MAX);
    |     trajectory(3).max_vel = single(MPC_Z_VEL_MAX_DN);
    | end
    | 
    | end
  function ManualPosition_checkEkfResetCounters:
    | function ManualPosition_checkEkfResetCounters
    | 
    | if local_position.xy_reset_counter ~= reset_counter_xy_
    |     reset_counter_xy_ = local_position.xy_reset_counter;
    | end
    | 
    | if local_position.vxy_reset_counter ~= reset_counter_vxy_
    |     reset_counter_vxy_ = local_position.vxy_reset_counter;
    | end
    | 
    | if local_position.z_reset_counter ~= reset_counter_z_
    |     reset_counter_z_ = local_position.z_reset_counter;
    | end
    | 
    | if local_position.vz_reset_counter ~= reset_counter_vz_
    |     reset_counter_vz_ = local_position.vz_reset_counter;
    | end
    | 
    | if local_position.heading_reset_counter ~= reset_counter_heading_
    |     reset_counter_heading_ = local_position.heading_reset_counter;
    |     
    |     if isfinite(yaw_setpoint)
    |         yaw_setpoint = yaw_setpoint + local_position.delta_heading;
    |     end
    | end
    | 
    | end
  function ManualPosition_scaleSticks:
    | function ManualPosition_scaleSticks
    | % calculate yawspeed and velocity setpoints by sticks
    | 
    | % manual altitude scaleSticks
    | % Use stick input with deadzone, exponential curve and first order lpf for yawspeed
    | yawspeed_target = positions_expo_(4) * deg2rad(MPC_MAN_Y_MAX);
    | yawspeed_setpoint = applyYawspeedFilter4(yawspeed_target);
    | 
    | % Use sticks input with deadzone and exponential curve for vertical velocity
    | if stick_positions_(3) > 0
    |     vel_max_z = constraints.speed_down;
    | else
    |     vel_max_z = constraints.speed_up;
    | end
    | velocity_setpoint(3) = vel_max_z * positions_expo_(3);
    | 
    | % Constrain length of stick inputs to 1 for xy
    | stick_xy = [positions_expo_(1), positions_expo_(2)];
    | magnitude = constrain(norm(stick_xy), 0, 1);
    | if magnitude > eps
    |     stick_xy = stick_xy / norm(stick_xy) * magnitude;
    | end
    | 
    | max_speed_from_estimator = local_position.vxy_max;
    | if isfinite(max_speed_from_estimator)
    |     velocity_scale = max(min(constraints.speed_xy, max_speed_from_estimator), single(0.3));
    | else
    |     velocity_scale = constraints.speed_xy;
    | end
    | 
    | % scale velocity to its maximum limits
    | vel_sp_xy = stick_xy * velocity_scale;
    | % Rotate setpoint into local frame
    | vel_sp_xy = rotateIntoHeadingFrame(vel_sp_xy);
    | 
    | velocity_setpoint(1) = vel_sp_xy(1);
    | velocity_setpoint(2) = vel_sp_xy(2);
    | end
    | 
    | %% 
    | function y = applyYawspeedFilter4(u)
    | 
    | persistent yawspeed_filter_state
    | if isempty(yawspeed_filter_state)
    |     yawspeed_filter_state = single(0);
    | end
    | 
    | den = max(MPC_MAN_Y_TAU + deltatime_, single(0.001));
    | alpha = deltatime_ / den;
    | yawspeed_filter_state = (1 - alpha) * yawspeed_filter_state + alpha * u;
    | 
    | y = yawspeed_filter_state;
    | end
  function ManualPosition_updateSetpoints:
    | function ManualPosition_updateSetpoints
    | 
    | persistent man_pos_reset_counter
    | if isempty(man_pos_reset_counter)
    |     man_pos_reset_counter = uint8(0);
    | end
    | 
    | ManualAltitude_updateSetpoints
    | acceleration_setpoint = [single(nan); single(nan); single(nan)];
    | 
    | % check for position lock XY
    | vel_xy_norm = norm([velocity_(1), velocity_(2)]);
    | apply_brake = (norm([velocity_setpoint(1), velocity_setpoint(2)]) < eps);
    | stopped = ((MPC_HOLD_MAX_XY < eps) || (vel_xy_norm < MPC_HOLD_MAX_XY));
    | 
    | if apply_brake && stopped && ~isfinite(position_setpoint(1))
    |     position_setpoint(1) = position_(1);
    |     position_setpoint(2) = position_(2);
    |     
    | elseif isfinite(position_setpoint(1)) && apply_brake
    |     if local_position.xy_reset_counter ~= man_pos_reset_counter
    |         position_setpoint(1) = position_(1);
    |         position_setpoint(2) = position_(2);
    |         man_pos_reset_counter = local_position.xy_reset_counter;
    |     end
    |     
    | else
    |     position_setpoint(1) = single(nan);
    |     position_setpoint(2) = single(nan);
    | end
    | 
    | % check if an external yaw handler is active and if yes, let it update the yaw setpoints
    | if ~isempty(fieldnames(weathervane_yaw_handler)) && weathervane_yaw_handler.is_active
    |     yaw_setpoint = single(nan);
    |     
    |     if isfinite(position_setpoint(1)) && isfinite(position_setpoint(2))
    |         yawspeed_setpoint = yawspeed_setpoint + get_weathervane_yawrate(weathervane_yaw_handler.dcm_z_sp_prev, weathervane_yaw_handler.yaw);
    |     end
    | end
    | 
    | end
  function ManualAltitude_updateSetpoints:
    | function ManualAltitude_updateSetpoints
    | % calculate acc_sp_XY and pos_sp_Z
    | 
    | % get yaw setpoint
    | if abs(yawspeed_setpoint) > 0.001
    |     yaw_setpoint = single(nan);
    | else
    |     yaw_setpoint = IsFinite(yaw_setpoint, yaw_);
    | end
    | 
    | sp = [stick_positions_(1), stick_positions_(2)];
    | sp = man_input_filter4(sp);
    | sp = rotateIntoHeadingFrame(sp);
    | if norm(sp) > 1
    |     sp = sp / norm(sp);
    | end
    | 
    | a = sp * tan(deg2rad(MPC_MAN_TILT_MAX)) * CONSTANTS_ONE_G;
    | acceleration_setpoint(1) = a(1);
    | acceleration_setpoint(2) = a(2);
    | 
    | updateAltitudeLock4;
    | 
    | % respectGroundSlowdown——limit speed gradually within the altitudes MPC_LAND_ALT1 and MPC_LAND_ALT2
    | if isfinite(dist_to_ground_)
    |     limit_down = gradual(dist_to_ground_, MPC_LAND_ALT2, MPC_LAND_ALT1, MPC_LAND_SPEED, constraints.speed_down);
    |     limit_up = gradual(dist_to_ground_, MPC_LAND_ALT2, MPC_LAND_ALT1, MPC_TKO_SPEED, constraints.speed_up);
    |     velocity_setpoint(3) = constrain(velocity_setpoint(3), -limit_up, limit_down);
    | end
    | 
    | end
    | 
    | %% 
    | function y = man_input_filter4(u)
    | 
    | persistent alpha filter_state
    | if isempty(alpha)
    |     alpha = single(1);
    | end
    | if isempty(filter_state)
    |     filter_state = [single(0), single(0)];
    | end
    | 
    | denominator = MC_MAN_TILT_TAU + deltatime_;
    | if denominator > eps
    |     alpha = deltatime_ / denominator;
    | end
    | 
    | filter_state = (1 - alpha) * filter_state + alpha * u;
    | y = filter_state;
    | 
    | end
    | 
    | %% 
    | function updateAltitudeLock4
    | 
    | persistent terrain_hold terrain_follow dist_to_ground_lock man_alt_reset_counter
    | if isempty(terrain_hold)
    |     terrain_hold = false;
    | end
    | if isempty(terrain_follow)
    |     terrain_follow = false;
    | end
    | if isempty(dist_to_ground_lock)
    |     dist_to_ground_lock = single(nan);
    | end
    | if isempty(man_alt_reset_counter)
    |     man_alt_reset_counter = uint8(0);
    | end
    | 
    | % Check if user wants to break
    | apply_brake = (abs(positions_expo_(3)) <= eps);
    | % Check if vehicle has stopped
    | stopped = ((MPC_HOLD_MAX_Z < eps) || (abs(velocity_(3)) < MPC_HOLD_MAX_Z));
    | 
    | if MPC_ALT_MODE == 2
    | % control height relative to ground
    |     spd_xy = norm([velocity_(1), velocity_(2)]);
    |     stick_xy = norm([positions_expo_(1), positions_expo_(2)]);
    |     stick_input = (stick_xy > 0.001);
    |     
    |     if terrain_hold
    |         too_fast = (spd_xy > MPC_HOLD_MAX_XY);
    |         
    |         if stick_input || too_fast || ~isfinite(dist_to_bottom_)
    |             terrain_hold = false;
    |             terrain_follow = false;
    |             
    |             if isfinite(dist_to_ground_lock) && isfinite(dist_to_bottom_)
    |                 position_setpoint(3) = position_(3) - (dist_to_ground_lock - dist_to_bottom_);
    |             else
    |                 position_setpoint(3) = position_(3);
    |             end
    |         end
    |     else
    |         not_moving = (spd_xy < 0.5 * MPC_HOLD_MAX_XY);
    |         
    |         if ~stick_input && not_moving && isfinite(dist_to_bottom_)
    |             terrain_hold = true;
    |             terrain_follow = true;
    |             
    |             if isfinite(position_setpoint(3))
    |                 dist_to_ground_lock = dist_to_bottom_ - (position_setpoint(3) - position_(3));
    |             end
    |         end
    |     end
    | end
    | 
    | if (MPC_ALT_MODE == 1 || terrain_follow) && isfinite(dist_to_bottom_)
    | % control height relative to estimated distance to ground
    | 
    |     dist_to_ground_lock = terrainFollowing(apply_brake, stopped, dist_to_ground_lock);
    |     respectMaxAltitude;
    |     
    | else
    | % control height relative to the earth frame origin
    | 
    |     if apply_brake && stopped && ~isfinite(position_setpoint(3))
    |         % lock altitude
    |         position_setpoint(3) = position_(3);
    |         
    |         if isfinite(dist_to_bottom_) && (dist_to_bottom_ < min_distance_to_ground_)
    |             dist_to_ground_lock = terrainFollowing(apply_brake, stopped, dist_to_ground_lock);
    |         else
    |             dist_to_ground_lock = single(nan);
    |         end
    |         
    |     elseif isfinite(position_setpoint(3)) && apply_brake
    |         % altitude is locked but check if a reset event has happened
    |         if local_position.z_reset_counter ~= man_alt_reset_counter
    |             position_setpoint(3) = position_(3);
    |             man_alt_reset_counter = local_position.z_reset_counter;
    |         end
    |         
    |     else
    |         position_setpoint(3) = single(nan);
    |         respectMaxAltitude
    |     end
    | end
    | 
    | end
  function takeoff_reactivate:
    | function takeoff_reactivate
    | 
    | if takeoff_state < uint8(PX4_TAKEOFF_STATUS.TAKEOFF_STATE_RAMPUP)
    |     FlightTask_activate;
    | end
    | 
    | end
  function out = switchTask:
    | function out = switchTask
    | out = true;
    | 
    | if task_ ~= task_last_
    |     % getPositionSetpoint
    |     last_setpoint.x = position_setpoint(1);
    |     last_setpoint.y = position_setpoint(2);
    |     last_setpoint.z = position_setpoint(3);
    | 
    |     last_setpoint.vx = velocity_setpoint(1);
    |     last_setpoint.vy = velocity_setpoint(2);
    |     last_setpoint.vz = velocity_setpoint(3);
    | 
    |     last_setpoint.yaw = yaw_setpoint;
    |     last_setpoint.yawspeed = yawspeed_setpoint;
    | 
    |     last_setpoint.acceleration = acceleration_setpoint;
    |     last_setpoint.jerk = jerk_setpoint;
    |     last_setpoint.thrust = [single(nan); single(nan); single(nan)];
    | 
    |     % updateInitialize
    |     FlightTask_updateInitialize;
    |     flag_init = Sticks_checkAndSetStickInputs && isfinite(yaw_) &&...
    |             isfinite(position_(1)) && isfinite(position_(2)) && isfinite(position_(3)) &&...
    |             isfinite(velocity_(1)) && isfinite(velocity_(2)) && isfinite(velocity_(3));
    | 
    |     % active
    |     FlightTaskManualAltitude_activate;
    | 
    |     constraints.speed_xy = min(constraints.speed_xy, MPC_VEL_MANUAL);
    |     position_setpoint(1) = position_(1);
    |     position_setpoint(2) = position_(2);
    |     velocity_setpoint(1) = single(0);
    |     velocity_setpoint(2) = single(0);
    |     velocity_scale = constraints.speed_xy;
    | 
    |     out = flag_init;
    | end
    | 
    | end
  function ManualPositionSmoothVel_checkEkfResetCounters:
    | function ManualPositionSmoothVel_checkEkfResetCounters
    | 
    | if local_position.xy_reset_counter ~= reset_counter_xy_
    |     reset_counter_xy_ = local_position.xy_reset_counter;
    |     
    |     trajectory(1).state_x = position_(1);
    |     trajectory(1).state_init_x = position_(1);
    |     trajectory(2).state_x = position_(2);
    |     trajectory(2).state_init_x = position_(2);
    |     position_estimate(1) = position_(1);
    |     position_estimate(2) = position_(2);
    |     
    |     if position_lock_active_xy
    |         position_setpoint_locked(1) = position_(1);
    |         position_setpoint_locked(2) = position_(2);
    |     end
    | end
    | 
    | if local_position.vxy_reset_counter ~= reset_counter_vxy_
    |     reset_counter_vxy_ = local_position.vxy_reset_counter;
    |     
    |     trajectory(1).state_v = velocity_(1);
    |     trajectory(1).state_init_v = velocity_(1);
    |     trajectory(2).state_v = velocity_(2);
    |     trajectory(2).state_init_v = velocity_(2);
    | end
    | 
    | if local_position.z_reset_counter ~= reset_counter_z_
    |     reset_counter_z_ = local_position.z_reset_counter;
    |     
    |     trajectory(3).state_x = position_(3);
    |     trajectory(3).state_init_x = position_(3);
    |     position_estimate(3) = position_(3);
    |     
    |     if position_lock_active_z
    |         position_setpoint_locked(3) = position_(3);
    |     end
    | end
    | 
    | if local_position.vz_reset_counter ~= reset_counter_vz_
    |     reset_counter_vz_ = local_position.vz_reset_counter;
    |     
    |     trajectory(3).state_v = velocity_(3);
    |     trajectory(3).state_init_v = velocity_(3);
    | end
    | 
    | if local_position.heading_reset_counter ~= reset_counter_heading_
    |     reset_counter_heading_ = local_position.heading_reset_counter;
    |     
    |     if isfinite(yaw_setpoint)
    |         yaw_setpoint = yaw_setpoint + local_position.delta_heading;
    |     end
    | end 
    | 
    | end
  function ManualPositionSmoothVel_scaleSticks:
    | function ManualPositionSmoothVel_scaleSticks
    | % calculate yawspeed and velocity setpoints by sticks
    | 
    | % manual altitude scaleSticks
    | % Use stick input with deadzone, exponential curve and first order lpf for yawspeed
    | yawspeed_target = positions_expo_(4) * deg2rad(MPC_MAN_Y_MAX);
    | yawspeed_setpoint = applyYawspeedFilter3(yawspeed_target);
    | 
    | % Use sticks input with deadzone and exponential curve for vertical velocity
    | if stick_positions_(3) > 0
    |     vel_max_z = constraints.speed_down;
    | else
    |     vel_max_z = constraints.speed_up;
    | end
    | velocity_setpoint(3) = vel_max_z * positions_expo_(3);
    | 
    | % Constrain length of stick inputs to 1 for xy
    | stick_xy = [positions_expo_(1), positions_expo_(2)];
    | magnitude = constrain(norm(stick_xy), 0, 1);
    | if magnitude > eps
    |     stick_xy = stick_xy / norm(stick_xy) * magnitude;
    | end
    | 
    | max_speed_from_estimator = local_position.vxy_max;
    | if isfinite(max_speed_from_estimator)
    |     velocity_scale = max(min(constraints.speed_xy, max_speed_from_estimator), single(0.3));
    | else
    |     velocity_scale = constraints.speed_xy;
    | end
    | 
    | % scale velocity to its maximum limits
    | vel_sp_xy = stick_xy * velocity_scale;
    | % Rotate setpoint into local frame
    | vel_sp_xy = rotateIntoHeadingFrame(vel_sp_xy);
    | 
    | velocity_setpoint(1) = vel_sp_xy(1);
    | velocity_setpoint(2) = vel_sp_xy(2);
    | end
    | 
    | %% 
    | function y = applyYawspeedFilter3(u)
    | 
    | persistent yawspeed_filter_state
    | if isempty(yawspeed_filter_state)
    |     yawspeed_filter_state = single(0);
    | end
    | 
    | den = max(MPC_MAN_Y_TAU + deltatime_, single(0.001));
    | alpha = deltatime_ / den;
    | yawspeed_filter_state = (1 - alpha) * yawspeed_filter_state + alpha * u;
    | 
    | y = yawspeed_filter_state;
    | end
  function ManualPositionSmoothVel_updateSetpoints:
    | function ManualPositionSmoothVel_updateSetpoints
    | 
    | persistent man_pos_reset_counter
    | if isempty(man_pos_reset_counter)
    |     man_pos_reset_counter = uint8(0);
    | end
    | 
    | % updateTrajConstraints
    | trajectory(1).max_jerk = MPC_JERK_MAX;
    | trajectory(2).max_jerk = MPC_JERK_MAX;
    | trajectory(3).max_jerk = MPC_JERK_MAX;
    | trajectory(1).max_accel = MPC_ACC_HOR_MAX;
    | trajectory(2).max_accel = MPC_ACC_HOR_MAX;
    | trajectory(1).max_vel = constraints.speed_xy;
    | trajectory(2).max_vel = constraints.speed_xy;
    | 
    | % updateTrajCurrentPositionEstimate
    | position_estimate = position_;
    | 
    | % manual position updateSetpoints
    | ManualAltitude_updateSetpoints
    | acceleration_setpoint = [single(nan); single(nan); single(nan)];
    | 
    | % check for position lock
    | vel_xy_norm = norm([velocity_(1), velocity_(2)]);
    | apply_brake = (norm([velocity_setpoint(1), velocity_setpoint(2)]) < eps);
    | stopped = ((MPC_HOLD_MAX_XY < eps) || (vel_xy_norm < MPC_HOLD_MAX_XY));
    | 
    | if apply_brake && stopped && ~isfinite(position_setpoint(1))
    |     position_setpoint(1) = position_(1);
    |     position_setpoint(2) = position_(2);
    |     
    | elseif apply_brake && isfinite(position_setpoint(1))
    |     if local_position.xy_reset_counter ~= man_pos_reset_counter
    |         position_setpoint(1) = position_(1);
    |         position_setpoint(2) = position_(2);
    |         man_pos_reset_counter = local_position.xy_reset_counter;
    |     end
    |     
    | else
    |     position_setpoint(1) = single(nan);
    |     position_setpoint(2) = single(nan);
    | end
    | 
    | % check if an external yaw handler is active and if yes, let it update the yaw setpoints
    | if ~isempty(fieldnames(weathervane_yaw_handler)) && weathervane_yaw_handler.is_active
    |     yaw_setpoint = single(nan);
    |     
    |     if isfinite(position_setpoint(1)) && isfinite(position_setpoint(2))
    |         yawspeed_setpoint = yawspeed_setpoint + get_weathervane_yawrate(weathervane_yaw_handler.dcm_z_sp_prev, weathervane_yaw_handler.yaw);
    |     end
    | end
    | 
    | % 
    | updateTrajectories(velocity_setpoint);
    | 
    | % output
    | jerk_setpoint = [trajectory(1).state_j; trajectory(2).state_j; trajectory(3).state_j];
    | acceleration_setpoint = [trajectory(1).state_a; trajectory(2).state_a; trajectory(3).state_a];
    | velocity_setpoint = [trajectory(1).state_v; trajectory(2).state_v; trajectory(3).state_v];
    | position_setpoint = position_setpoint_locked;
    | 
    | end
    | 
    | %% 
    | function updateTrajectories(vel_target)
    | 
    | % update trajectories XY
    | for i = 1:1:2
    |     trajectory(i) = VelocitySmoothing_updateTraj(deltatime_, single(1), trajectory(i));
    | end
    | 
    | % check position lock XY
    | if (norm([trajectory(1).state_v, trajectory(2).state_v]) < 0.1) && (norm([trajectory(1).state_a, trajectory(2).state_a]) < 0.2) && (norm([vel_target(1), vel_target(2)]) <= eps)
    |     position_lock_active_xy = true;
    |     position_setpoint_locked(1) = trajectory(1).state_init_x;
    |     position_setpoint_locked(2) = trajectory(2).state_init_x;
    |     
    | else
    |     if position_lock_active_xy
    |         trajectory(1).state_init_v = velocity_setpoint_feedback_(1);
    |         trajectory(1).state_v = velocity_setpoint_feedback_(1);
    |         trajectory(2).state_init_v = velocity_setpoint_feedback_(2);
    |         trajectory(2).state_v = velocity_setpoint_feedback_(2);
    |         
    |         % reset position lock
    |         position_lock_active_xy = false;
    |         position_setpoint_locked(1) = single(nan);
    |         position_setpoint_locked(2) = single(nan);
    |     end
    |     
    |     trajectory(1).state_init_x = position_estimate(1);
    |     trajectory(1).state_x = position_estimate(1);
    |     trajectory(2).state_init_x = position_estimate(2);
    |     trajectory(2).state_x = position_estimate(2);
    | end
    | 
    | % update durations XY
    | for i = 1:1:2
    |     trajectory(i) = VelocitySmoothing_updateDurations(vel_target(i),trajectory(i));
    | end
    | % Synchronize XY trajectories to have the same total time. This is required to generate straight lines.
    | trajectory = VelocitySmoothing_timeSynchronization(trajectory, 2);
    | 
    | % update trajectories Z
    | trajectory(3) = VelocitySmoothing_updateTraj(deltatime_, single(1), trajectory(3));
    | 
    | % check position lock Z
    | if vel_target(3) < 0
    |     trajectory(3).max_accel = MPC_ACC_UP_MAX;
    |     trajectory(3).max_vel = constraints.speed_up;
    | else
    |     trajectory(3).max_accel = MPC_ACC_DOWN_MAX;
    |     trajectory(3).max_vel = constraints.speed_down;
    | end
    | 
    | if (abs(trajectory(3).state_v) < 0.1) && (abs(trajectory(3).state_a) < 0.2) && (abs(vel_target(3)) <= eps)
    |     position_lock_active_z = true;
    |     position_setpoint_locked(3) = trajectory(3).state_x;
    | else
    |     if position_lock_active_z
    |         trajectory(3).state_init_v = velocity_setpoint_feedback_(3);
    |         trajectory(3).state_v = velocity_setpoint_feedback_(3);
    |         
    |         position_lock_active_z = false;
    |         position_setpoint_locked(3) = single(nan);
    |     end
    |     trajectory(3).state_init_x = position_estimate(3);
    |     trajectory(3).state_x = position_estimate(3);
    | end
    | 
    | % update durations Z
    | trajectory(3) = VelocitySmoothing_updateDurations(vel_target(3),trajectory(3));
    | 
    | end
  function ManualAltitude_updateSetpoints:
    | function ManualAltitude_updateSetpoints
    | % calculate acc_sp_XY and pos_sp_Z
    | 
    | % get yaw setpoint
    | if abs(yawspeed_setpoint) > 0.001
    |     yaw_setpoint = single(nan);
    | else
    |     if (~isfinite(yaw_setpoint))
    |         yaw_setpoint = yaw_;
    |     end
    | end
    | 
    | sp = [stick_positions_(1), stick_positions_(2)];
    | sp = man_input_filter3(sp);
    | sp = rotateIntoHeadingFrame(sp);
    | if norm(sp) > 1
    |     sp = sp / norm(sp);
    | end
    | 
    | a = sp * tan(deg2rad(MPC_MAN_TILT_MAX)) * CONSTANTS_ONE_G;
    | acceleration_setpoint(1) = a(1);
    | acceleration_setpoint(2) = a(2);
    | 
    | updateAltitudeLock3;
    | 
    | % respectGroundSlowdown——limit speed gradually within the altitudes MPC_LAND_ALT1 and MPC_LAND_ALT2
    | if isfinite(dist_to_ground_)
    |     limit_down = gradual(dist_to_ground_, MPC_LAND_ALT2, MPC_LAND_ALT1, MPC_LAND_SPEED, constraints.speed_down);
    |     limit_up = gradual(dist_to_ground_, MPC_LAND_ALT2, MPC_LAND_ALT1, MPC_TKO_SPEED, constraints.speed_up);
    |     velocity_setpoint(3) = constrain(velocity_setpoint(3), -limit_up, limit_down);
    | end
    | 
    | end
    | 
    | %% 
    | function y = man_input_filter3(u)
    | 
    | persistent alpha filter_state
    | if isempty(alpha)
    |     alpha = single(1);
    | end
    | if isempty(filter_state)
    |     filter_state = [single(0), single(0)];
    | end
    | 
    | denominator = MC_MAN_TILT_TAU + deltatime_;
    | if denominator > eps
    |     alpha = deltatime_ / denominator;
    | end
    | 
    | filter_state = (1 - alpha) * filter_state + alpha * u;
    | y = filter_state;
    | 
    | end
    | 
    | %% 
    | function updateAltitudeLock3
    | 
    | persistent terrain_hold terrain_follow dist_to_ground_lock man_alt_reset_counter
    | if isempty(terrain_hold)
    |     terrain_hold = false;
    | end
    | if isempty(terrain_follow)
    |     terrain_follow = false;
    | end
    | if isempty(dist_to_ground_lock)
    |     dist_to_ground_lock = single(nan);
    | end
    | if isempty(man_alt_reset_counter)
    |     man_alt_reset_counter = uint8(0);
    | end
    | 
    | % Check if user wants to break
    | apply_brake = (abs(positions_expo_(3)) <= eps);
    | % Check if vehicle has stopped
    | stopped = ((MPC_HOLD_MAX_Z < eps) || (abs(velocity_(3)) < MPC_HOLD_MAX_Z));
    | 
    | if MPC_ALT_MODE == 2
    | % control height relative to ground
    |     spd_xy = norm([velocity_(1), velocity_(2)]);
    |     stick_xy = norm([positions_expo_(1), positions_expo_(2)]);
    |     stick_input = (stick_xy > 0.001);
    |     
    |     if terrain_hold
    |         too_fast = (spd_xy > MPC_HOLD_MAX_XY);
    |         
    |         if stick_input || too_fast || ~isfinite(dist_to_bottom_)
    |             terrain_hold = false;
    |             terrain_follow = false;
    |             
    |             if isfinite(dist_to_ground_lock) && isfinite(dist_to_bottom_)
    |                 position_setpoint(3) = position_(3) - (dist_to_ground_lock - dist_to_bottom_);
    |             else
    |                 position_setpoint(3) = position_(3);
    |             end
    |         end
    |     else
    |         not_moving = (spd_xy < 0.5 * MPC_HOLD_MAX_XY);
    |         
    |         if ~stick_input || not_moving || isfinite(dist_to_bottom_)
    |             terrain_hold = true;
    |             terrain_follow = true;
    |             
    |             if isfinite(position_setpoint(3))
    |                 dist_to_ground_lock = dist_to_bottom_ - (position_setpoint(3) - position_(3));
    |             end
    |         end
    |     end
    | end
    | 
    | if (MPC_ALT_MODE == 1 || terrain_follow) && isfinite(dist_to_bottom_)
    | % control height relative to estimated distance to ground
    |     
    |     dist_to_ground_lock = terrainFollowing(apply_brake, stopped, dist_to_ground_lock);
    |     respectMaxAltitude;
    |     
    | else
    | % control height relative to the earth frame origin
    |     
    |     if apply_brake && stopped && ~isfinite(position_setpoint(3))
    |         % lock altitude 
    |         position_setpoint(3) = position_(3);
    |         
    |         if isfinite(dist_to_bottom_) && (dist_to_bottom_ < min_distance_to_ground_)
    |             dist_to_ground_lock = terrainFollowing(apply_brake, stopped, dist_to_ground_lock);
    |         else
    |             dist_to_ground_lock = single(nan);
    |         end
    |         
    |     elseif isfinite(position_setpoint(3)) && apply_brake
    |         % altitude is locked but check if a reset event has happened
    |         if local_position.z_reset_counter ~= man_alt_reset_counter
    |             position_setpoint(3) = position_(3);
    |             man_alt_reset_counter = local_position.z_reset_counter;
    |         end
    |         
    |     else
    |         position_setpoint(3) = single(nan);
    |         respectMaxAltitude
    |     end
    | end
    | 
    | end
  function takeoff_reactivate:
    | function takeoff_reactivate
    | 
    | if takeoff_state < uint8(PX4_TAKEOFF_STATUS.TAKEOFF_STATE_RAMPUP)
    |     FlightTask_activate
    |     
    |     for i=1:1:3
    |         trajectory(i).state_j = single(0);
    |         trajectory(i).state_a = single(0);
    |         trajectory(i).state_v = velocity_(i);
    |         trajectory(i).state_x = position_(i);
    |         if i==3
    |             trajectory(i).state_v = single(0);
    |         end
    |        
    |         trajectory(i).state_init_j = trajectory(i).state_j;
    |         trajectory(i).state_init_a = trajectory(i).state_a;
    |         trajectory(i).state_init_v = trajectory(i).state_v;
    |         trajectory(i).state_init_x = trajectory(i).state_x;
    |         
    |         position_setpoint_locked(i) = single(nan);
    |     end
    |     
    |     position_lock_active_xy = false;
    |     position_lock_active_z = false;
    | end
    | 
    | end
  function result = switchTask:
    | function result = switchTask()
    | 
    | if (task_ == task_last_)
    |     % 飞行模式未改变
    |     result = true;
    | else
    |     % 飞行模式已改变
    |     % 获取当前的position setpoint为最新的飞行模式做准备
    |     last_setpoint.timestamp = uint64(getSimulationTime * 1e+6);
    |     
    |     last_setpoint.x = position_setpoint(1);
    |     last_setpoint.y = position_setpoint(2);
    |     last_setpoint.z = position_setpoint(3);
    |     
    |     last_setpoint.vx = velocity_setpoint(1);
    |     last_setpoint.vy = velocity_setpoint(2);
    |     last_setpoint.vz = velocity_setpoint(3);
    |     
    |     last_setpoint.yaw = yaw_setpoint;
    |     last_setpoint.yawspeed = yawspeed_setpoint;
    |     
    |     last_setpoint.acceleration = acceleration_setpoint;
    |     last_setpoint.jerk = jerk_setpoint;
    |     last_setpoint.thrust = single([nan; nan; nan]);
    |     
    |     % 记录ekf_resetcounters
    |     
    |     %% updateInitialize: 记录模式初始时间和输入数据
    |     mode_action.FlightTask_updateInitialize();
    |     flag_init = mode_action.Sticks_checkAndSetStickInputs && ...
    |         isfinite(position_(3)) && isfinite(velocity_(3)) && isfinite(yaw_);
    |     
    |     %% manual position smooth vel active
    |     % 所有来自高度模式的要求仍然必须保持(all requirements from altitude-mode still have to
    |     % hold)
    |     mode_action.FlightTaskManualAltitude_activate();
    |     
    |     % 设置水平速度限幅
    |     constraints.speed_xy = min(constraints.speed_xy, MPC_VEL_MANUAL);
    |     position_setpoint(1) = position_(1);
    |     position_setpoint(2) = position_(2);
    |     velocity_setpoint(1) = single(0.0);
    |     velocity_setpoint(2) = single(0.0);
    |     velocity_scale       = constraints.speed_xy;
    |     
    |     % 检查上次飞行任务是否提供setpoints(Check if the previous FlightTask provided
    |     % setpoints)
    |     accel_prev = last_setpoint.acceleration;
    |     vel_prev   = [last_setpoint.vx, last_setpoint.vy, last_setpoint.vz];
    |     pos_prev   = [last_setpoint.x, last_setpoint.y, last_setpoint.z];
    |     
    |     pos_curr   = [local_position.x, local_position.y, local_position.z];
    |     vel_curr   = [local_position.vx, local_position.vy, local_position.vz];
    |     
    |     for i = 1:3
    |         % If the position setpoint is unknown, set to the current postion
    |         if (~isfinite(pos_prev(i)))
    |             pos_prev(i) = pos_curr(i);
    |         end
    |         
    |         % If the velocity setpoint is unknown, set to the current velocity
    |         if (~isfinite(vel_prev(i)))
    |             vel_prev(i) = vel_curr(i);
    |         end
    |         
    |         % No acceleration estimate available, set to zero if the setpoint is NAN
    |         if (~isfinite(accel_prev(i)))
    |             accel_prev(i) = single(0.0);
    |         end
    |     end
    |     
    |     % smooth_xy and smooth_z
    |     % j: jerk; 
    |     % a: acceleration; 
    |     % v: velocity; 
    |     % x: position;
    |     for i = 1:3
    |         trajectory(i).state_j = single(0.0);
    |         trajectory(i).state_a = accel_prev(i);
    |         trajectory(i).state_v = vel_prev(i);
    |         trajectory(i).state_x = pos_prev(i);
    |         
    |         trajectory(i).state_init_x = trajectory(i).state_x;
    |         trajectory(i).state_init_v = trajectory(i).state_v;
    |         trajectory(i).state_init_a = trajectory(i).state_a;
    |         trajectory(i).state_init_j = trajectory(i).state_j;
    |     end
    |     
    |     position_lock_active_xy  = false;
    |     position_lock_active_z   = false;
    |     position_setpoint_locked = single([nan; nan; nan]);
    |     
    |     result = flag_init;
    | end
    | 
    | end
  function ManualAltitude_checkEkfResetCounters:
    | function ManualAltitude_checkEkfResetCounters
    | 
    | if local_position.xy_reset_counter ~= reset_counter_xy_
    |     reset_counter_xy_ = local_position.xy_reset_counter;
    | end
    | 
    | if local_position.vxy_reset_counter ~= reset_counter_vxy_
    |     reset_counter_vxy_ = local_position.vxy_reset_counter;
    | end
    | 
    | if local_position.z_reset_counter ~= reset_counter_z_
    |     reset_counter_z_ = local_position.z_reset_counter;
    | end
    | 
    | if local_position.vz_reset_counter ~= reset_counter_vz_
    |     reset_counter_vz_ = local_position.vz_reset_counter;
    | end
    | 
    | if local_position.heading_reset_counter ~= reset_counter_heading_
    |     reset_counter_heading_ = local_position.heading_reset_counter;
    |     
    |     if isfinite(yaw_setpoint)
    |         yaw_setpoint = yaw_setpoint + local_position.delta_heading;
    |     end
    | end
    | 
    | end
  function ManualAltitude_scaleSticks:
    | function ManualAltitude_scaleSticks
    | % calculate yawspeed and velocity_Z setpoints by sticks
    | 
    | % Use stick input with deadzone, exponential curve and first order lpf for yawspeed
    | yawspeed_target = positions_expo_(4) * deg2rad(MPC_MAN_Y_MAX);
    | yawspeed_setpoint = applyYawspeedFilter2(yawspeed_target);
    | 
    | % Use sticks input with deadzone and exponential curve for vertical velocity
    | if stick_positions_(3) > 0
    |     vel_max_z = constraints.speed_down;
    | else
    |     vel_max_z = constraints.speed_up;
    | end
    | velocity_setpoint(3) = vel_max_z * positions_expo_(3);
    | 
    | end
    | 
    | %% 
    | function y = applyYawspeedFilter2(u)
    | 
    | persistent yawspeed_filter_state
    | if isempty(yawspeed_filter_state)
    |     yawspeed_filter_state = single(0);
    | end
    | 
    | den = max(MPC_MAN_Y_TAU + deltatime_, single(0.001));
    | alpha = deltatime_ / den;
    | yawspeed_filter_state = (1 - alpha) * yawspeed_filter_state + alpha * u;
    | 
    | y = yawspeed_filter_state;
    | end
  function ManualAltitude_updateSetpoints:
    | function ManualAltitude_updateSetpoints
    | % calculate acc_sp_XY and pos_sp_Z
    | 
    | % get yaw setpoint
    | if abs(yawspeed_setpoint) > 0.001
    |     yaw_setpoint = single(nan);
    | else
    |     yaw_setpoint = IsFinite(yaw_setpoint, yaw_);
    | end
    | 
    | sp = [stick_positions_(1), stick_positions_(2)];
    | sp = man_input_filter2(sp);
    | sp = rotateIntoHeadingFrame(sp);
    | if norm(sp) > 1
    |     sp = sp / norm(sp);
    | end
    | 
    | a = sp * tan(deg2rad(MPC_MAN_TILT_MAX)) * CONSTANTS_ONE_G;
    | acceleration_setpoint(1) = a(1);
    | acceleration_setpoint(2) = a(2);
    | 
    | updateAltitudeLock2;
    | 
    | % respectGroundSlowdown——limit speed gradually within the altitudes MPC_LAND_ALT1 and MPC_LAND_ALT2
    | if isfinite(dist_to_ground_)
    |     limit_down = gradual(dist_to_ground_, MPC_LAND_ALT2, MPC_LAND_ALT1, MPC_LAND_SPEED, constraints.speed_down);
    |     limit_up = gradual(dist_to_ground_, MPC_LAND_ALT2, MPC_LAND_ALT1, MPC_TKO_SPEED, constraints.speed_up);
    |     velocity_setpoint(3) = constrain(velocity_setpoint(3), -limit_up, limit_down);
    | end
    | 
    | end
    | 
    | %% 
    | function y = man_input_filter2(u)
    | 
    | persistent alpha filter_state
    | if isempty(alpha)
    |     alpha = single(1);
    | end
    | if isempty(filter_state)
    |     filter_state = [single(0), single(0)];
    | end
    | 
    | denominator = MC_MAN_TILT_TAU + deltatime_;
    | if denominator > eps
    |     alpha = deltatime_ / denominator;
    | end
    | 
    | filter_state = (1 - alpha) * filter_state + alpha * u;
    | y = filter_state;
    | 
    | end
    | 
    | %% 
    | function updateAltitudeLock2
    | 
    | persistent terrain_hold terrain_follow dist_to_ground_lock man_alt_reset_counter
    | if isempty(terrain_hold)
    |     terrain_hold = false;
    | end
    | if isempty(terrain_follow)
    |     terrain_follow = false;
    | end
    | if isempty(dist_to_ground_lock)
    |     dist_to_ground_lock = single(nan);
    | end
    | if isempty(man_alt_reset_counter)
    |     man_alt_reset_counter = uint8(0);
    | end
    | 
    | % Check if user wants to break
    | apply_brake = (abs(positions_expo_(3)) <= eps);
    | % Check if vehicle has stopped
    | stopped = ((MPC_HOLD_MAX_Z < eps) || (abs(velocity_(3)) < MPC_HOLD_MAX_Z));
    | 
    | if MPC_ALT_MODE == 2
    | % control height relative to ground
    |     spd_xy = norm([velocity_(1), velocity_(2)]);
    |     stick_xy = norm([positions_expo_(1), positions_expo_(2)]);
    |     stick_input = (stick_xy > 0.001);
    |     
    |     if terrain_hold
    |         too_fast = (spd_xy > MPC_HOLD_MAX_XY);
    |         
    |         if stick_input || too_fast || ~isfinite(dist_to_bottom_)
    |             terrain_hold = false;
    |             terrain_follow = false;
    |             
    |             if isfinite(dist_to_ground_lock) && isfinite(dist_to_bottom_)
    |                 position_setpoint(3) = position_(3) - (dist_to_ground_lock - dist_to_bottom_);
    |             else
    |                 position_setpoint(3) = position_(3);
    |             end
    |         end
    |     else
    |         not_moving = (spd_xy < 0.5 * MPC_HOLD_MAX_XY);
    |         
    |         if ~stick_input || not_moving || isfinite(dist_to_bottom_)
    |             terrain_hold = true;
    |             terrain_follow = true;
    |             
    |             if isfinite(position_setpoint(3))
    |                 dist_to_ground_lock = dist_to_bottom_ - (position_setpoint(3) - position_(3));
    |             end
    |         end
    |     end
    | end
    | 
    | if (MPC_ALT_MODE == 1 || terrain_follow) && isfinite(dist_to_bottom_)
    | % control height relative to estimated distance to ground
    |     
    |     dist_to_ground_lock = terrainFollowing(apply_brake, stopped, dist_to_ground_lock);
    |     respectMaxAltitude;
    |     
    | else
    | % control height relative to the earth frame origin
    |     
    |     if apply_brake && stopped && ~isfinite(position_setpoint(3))
    |         % lock altitude
    |         position_setpoint(3) = position_(3);
    |         
    |         if isfinite(dist_to_bottom_) && (dist_to_bottom_ < min_distance_to_ground_)
    |             dist_to_ground_lock = terrainFollowing(apply_brake, stopped, dist_to_ground_lock);
    |         else
    |             dist_to_ground_lock = single(nan);
    |         end
    |         
    |     elseif isfinite(position_setpoint(3)) && apply_brake
    |         % altitude is locked but check if a reset event has happened
    |         if local_position.z_reset_counter ~= man_alt_reset_counter
    |             position_setpoint(3) = position_(3);
    |             man_alt_reset_counter = local_position.z_reset_counter;
    |         end
    |         
    |     else
    |         position_setpoint(3) = single(nan);
    |         respectMaxAltitude
    |     end
    | end
    | 
    | end
  function takeoff_reactivate:
    | function takeoff_reactivate
    | 
    | if takeoff_state < uint8(PX4_TAKEOFF_STATUS.TAKEOFF_STATE_RAMPUP)
    |     FlightTask_activate;
    | end
    | 
    | end
  function result = switchTask:
    | function result = switchTask
    | 
    | result = true;
    | 
    | if task_ ~= task_last_
    |      % getPositionSetpoint
    |     last_setpoint.x = position_setpoint(1);
    |     last_setpoint.y = position_setpoint(2);
    |     last_setpoint.z = position_setpoint(3);
    | 
    |     last_setpoint.vx = velocity_setpoint(1);
    |     last_setpoint.vy = velocity_setpoint(2);
    |     last_setpoint.vz = velocity_setpoint(3);
    | 
    |     last_setpoint.yaw = yaw_setpoint;
    |     last_setpoint.yawspeed = yawspeed_setpoint;
    | 
    |     last_setpoint.acceleration = acceleration_setpoint;
    |     last_setpoint.jerk = jerk_setpoint;
    |     last_setpoint.thrust = single([nan; nan; nan]);
    | 
    |     % update initialize
    |     FlightTask_updateInitialize();
    |     flag_init = Sticks_checkAndSetStickInputs && isfinite(position_(3)) && isfinite(velocity_(3)) && isfinite(yaw_);
    | 
    |     % active
    |     FlightTaskManualAltitude_activate;
    |     result = flag_init;
    | end
    | 
    | end
  function ManualAltitudeSmoothVel_checkEkfResetCounters:
    | function ManualAltitudeSmoothVel_checkEkfResetCounters()
    | 
    | if local_position.xy_reset_counter ~= reset_counter_xy_
    |     reset_counter_xy_ = local_position.xy_reset_counter;
    | end
    | 
    | if local_position.vxy_reset_counter ~= reset_counter_vxy_
    |     reset_counter_vxy_ = local_position.vxy_reset_counter;
    | end
    | 
    | if local_position.z_reset_counter ~= reset_counter_z_
    |     reset_counter_z_ = local_position.z_reset_counter;
    |     
    |     trajectory.state_x = position_(3);
    |     trajectory.state_init_x = position_(3);
    |     position_estimate = position_(3);
    |     
    |     if position_lock_active_z
    |         position_setpoint_locked = position_(3);
    |     end
    | end
    | 
    | if local_position.vz_reset_counter ~= reset_counter_vz_
    |     reset_counter_vz_ = local_position.vz_reset_counter;
    |     
    |     trajectory.state_v = velocity_(3);
    |     trajectory.state_init_v = velocity_(3);
    | end
    | 
    | if local_position.heading_reset_counter ~= reset_counter_heading_
    |     reset_counter_heading_ = local_position.heading_reset_counter;
    |     
    |     if isfinite(yaw_setpoint)
    |         yaw_setpoint = yaw_setpoint + local_position.delta_heading;
    |     end
    | end
    | 
    | end
  function ManualAltitudeSmoothVel_scaleSticks:
    | function ManualAltitudeSmoothVel_scaleSticks()
    | % calculate yawspeed and velocity_Z setpoints by sticks
    | 
    | % Use stick input with deadzone, exponential curve and first order lpf for yawspeed
    | yawspeed_target = positions_expo_(4) * deg2rad(MPC_MAN_Y_MAX);
    | yawspeed_setpoint = applyYawspeedFilter1(yawspeed_target);
    | 
    | % Use sticks input with deadzone and exponential curve for vertical velocity
    | if stick_positions_(3) > 0
    |     vel_max_z = constraints.speed_down;
    | else
    |     vel_max_z = constraints.speed_up;
    | end
    | velocity_setpoint(3) = vel_max_z * positions_expo_(3);
    | 
    | end
    | 
    | %% 
    | function result = applyYawspeedFilter1(input)
    | 
    | persistent yawspeed_filter_state
    | 
    | if (isempty(yawspeed_filter_state))
    |     yawspeed_filter_state = single(0);
    | end
    | 
    | den = max(MPC_MAN_Y_TAU + deltatime_, single(0.001));
    | alpha = deltatime_ / den;
    | 
    | yawspeed_filter_state = (1 - alpha) * yawspeed_filter_state + alpha * input;
    | 
    | result = yawspeed_filter_state;
    | 
    | end
  function ManualAltitudeSmoothVel_updateSetpoints:
    | function ManualAltitudeSmoothVel_updateSetpoints
    | % updateTrajConstraints
    | trajectory.max_jerk = MPC_JERK_MAX;
    | position_estimate = position_(3);
    | 
    | % get yaw setpoint, acc_sp_XY, un-smoothed altitude setpoint
    | ManualAltitude_updateSetpoints;
    | 
    | % update state
    | trajectory = VelocitySmoothing_updateTraj(deltatime_,single(1),trajectory);
    | 
    | % set max accel/vel
    | if velocity_setpoint(3) < 0
    |     trajectory.max_accel = MPC_ACC_UP_MAX;
    |     trajectory.max_vel = constraints.speed_up;
    | else
    |     trajectory.max_accel = MPC_ACC_DOWN_MAX;
    |     trajectory.max_vel = constraints.speed_down;
    | end
    | 
    | % lock or unlock altitude
    | if (abs(trajectory.state_v) < 0.1) && (abs(trajectory.state_a) < 0.2) && (abs(velocity_setpoint(3)) <= eps)
    |     position_lock_active_z = true;
    |     position_setpoint_locked = trajectory.state_x;
    | else
    |     if position_lock_active_z
    |         trajectory.state_init_v = velocity_setpoint_feedback_(3);
    |         trajectory.state_v = velocity_setpoint_feedback_(3);
    |         
    |         position_lock_active_z = false;
    |         position_setpoint_locked = single(nan);
    |     end
    |     trajectory.state_init_x = position_estimate;
    |     trajectory.state_x = position_estimate;
    | end
    | 
    | % update durations
    | trajectory = VelocitySmoothing_updateDurations(velocity_setpoint(3), trajectory);
    | 
    | % set output state
    | jerk_setpoint(3) = trajectory.state_j;
    | acceleration_setpoint(3) = trajectory.state_a;
    | velocity_setpoint(3) = trajectory.state_v;
    | position_setpoint(3) = position_setpoint_locked;
    | 
    | end
  function ManualAltitude_updateSetpoints:
    | function ManualAltitude_updateSetpoints
    | % calculate acc_sp_XY and pos_sp_Z
    | 
    | % get yaw setpoint
    | if abs(yawspeed_setpoint) > 0.001
    |     yaw_setpoint = single(nan);
    | else
    |     yaw_setpoint = IsFinite(yaw_setpoint, yaw_);
    | end
    | 
    | sp = [stick_positions_(1), stick_positions_(2)];
    | sp = man_input_filter1(sp);
    | sp = rotateIntoHeadingFrame(sp);
    | if norm(sp) > 1
    |     sp = sp / norm(sp);
    | end
    | 
    | a = sp * tan(deg2rad(MPC_MAN_TILT_MAX)) * CONSTANTS_ONE_G;
    | acceleration_setpoint(1) = a(1);
    | acceleration_setpoint(2) = a(2);
    | 
    | updateAltitudeLock1;
    | 
    | % respectGroundSlowdown——limit speed gradually within the altitudes MPC_LAND_ALT1 and MPC_LAND_ALT2
    | if isfinite(dist_to_ground_)
    |     limit_down = gradual(dist_to_ground_, MPC_LAND_ALT2, MPC_LAND_ALT1, MPC_LAND_SPEED, constraints.speed_down);
    |     limit_up = gradual(dist_to_ground_, MPC_LAND_ALT2, MPC_LAND_ALT1, MPC_TKO_SPEED, constraints.speed_up);
    |     velocity_setpoint(3) = constrain(velocity_setpoint(3), -limit_up, limit_down);
    | end
    | 
    | end
    | 
    | %% 
    | function y = man_input_filter1(u)
    | 
    | persistent alpha filter_state
    | if isempty(alpha)
    |     alpha = single(1);
    | end
    | if isempty(filter_state)
    |     filter_state = [single(0), single(0)];
    | end
    | 
    | denominator = MC_MAN_TILT_TAU + deltatime_;
    | if denominator > eps
    |     alpha = deltatime_ / denominator;
    | end
    | 
    | filter_state = (1 - alpha) * filter_state + alpha * u;
    | y = filter_state;
    | 
    | end
    | 
    | %% 
    | function updateAltitudeLock1
    | 
    | persistent terrain_hold terrain_follow dist_to_ground_lock man_alt_reset_counter
    | if isempty(terrain_hold)
    |     terrain_hold = false;
    | end
    | if isempty(terrain_follow)
    |     terrain_follow = false;
    | end
    | if isempty(dist_to_ground_lock)
    |     dist_to_ground_lock = single(nan);
    | end
    | if isempty(man_alt_reset_counter)
    |     man_alt_reset_counter = uint8(0);
    | end
    | 
    | % Check if user wants to break
    | apply_brake = (abs(positions_expo_(3)) <= eps);
    | % Check if vehicle has stopped
    | stopped = ((MPC_HOLD_MAX_Z < eps) || (abs(velocity_(3)) < MPC_HOLD_MAX_Z));
    | 
    | if MPC_ALT_MODE == 2
    | % control height relative to ground
    |     spd_xy = norm([velocity_(1), velocity_(2)]);
    |     stick_xy = norm([positions_expo_(1), positions_expo_(2)]);
    |     stick_input = (stick_xy > 0.001);
    |     
    |     if terrain_hold
    |         too_fast = (spd_xy > MPC_HOLD_MAX_XY);
    |         
    |         if stick_input || too_fast || ~isfinite(dist_to_bottom_)
    |             terrain_hold = false;
    |             terrain_follow = false;
    |             
    |             if isfinite(dist_to_ground_lock) && isfinite(dist_to_bottom_)
    |                 position_setpoint(3) = position_(3) - (dist_to_ground_lock - dist_to_bottom_);
    |             else
    |                 position_setpoint(3) = position_(3);
    |             end
    |         end
    |     else
    |         not_moving = (spd_xy < 0.5 * MPC_HOLD_MAX_XY);
    |         
    |         if ~stick_input || not_moving || isfinite(dist_to_bottom_)
    |             terrain_hold = true;
    |             terrain_follow = true;
    |             
    |             if isfinite(position_setpoint(3))
    |                 dist_to_ground_lock = dist_to_bottom_ - (position_setpoint(3) - position_(3));
    |             end
    |         end
    |     end
    | end
    | 
    | if (MPC_ALT_MODE == 1 || terrain_follow) && isfinite(dist_to_bottom_)
    | % control height relative to estimated distance to ground
    | 
    |     dist_to_ground_lock = terrainFollowing(apply_brake, stopped, dist_to_ground_lock);
    |     respectMaxAltitude;
    |     
    | else
    | % control height relative to the earth frame origin
    |     
    |     if apply_brake && stopped && ~isfinite(position_setpoint(3))
    |         % lock altitude
    |         position_setpoint(3) = position_(3);
    |         
    |         if isfinite(dist_to_bottom_) && (dist_to_bottom_ < min_distance_to_ground_)
    |             dist_to_ground_lock = terrainFollowing(apply_brake, stopped, dist_to_ground_lock);
    |         else
    |             dist_to_ground_lock = single(nan);
    |         end
    |         
    |     elseif isfinite(position_setpoint(3)) && apply_brake
    |         % altitude is locked but check if a reset event has happened
    |         if local_position.z_reset_counter ~= man_alt_reset_counter
    |             position_setpoint(3) = position_(3);
    |             man_alt_reset_counter = local_position.z_reset_counter;
    |         end
    |         
    |     else
    |         position_setpoint(3) = single(nan);
    |         respectMaxAltitude
    |     end
    | end
    | 
    | end
  function takeoff_reactivate:
    | function takeoff_reactivate
    | 
    | if takeoff_state < uint8(PX4_TAKEOFF_STATUS.TAKEOFF_STATE_RAMPUP)
    |     FlightTask_activate;
    |     
    |     trajectory.state_j = single(0);
    |     trajectory.state_a = single(0);
    |     trajectory.state_v = single(0);
    |     trajectory.state_x = position_(3);
    |     
    |     trajectory.state_init_j = trajectory.state_j;
    |     trajectory.state_init_a = trajectory.state_a;
    |     trajectory.state_init_v = trajectory.state_v;
    |     trajectory.state_init_x = trajectory.state_x;
    |     
    |     position_lock_active_z = false;
    |     position_setpoint_locked = single(nan);
    | end
    | 
    | end
  function out = switchTask:
    | function out = switchTask()
    | out = true;
    | 
    | if task_ ~= task_last_
    |     % getPositionSetpoint
    |     last_setpoint.x = position_setpoint(1);
    |     last_setpoint.y = position_setpoint(2);
    |     last_setpoint.z = position_setpoint(3);
    | 
    |     last_setpoint.vx = velocity_setpoint(1);
    |     last_setpoint.vy = velocity_setpoint(2);
    |     last_setpoint.vz = velocity_setpoint(3);
    | 
    |     last_setpoint.yaw = yaw_setpoint;
    |     last_setpoint.yawspeed = yawspeed_setpoint;
    | 
    |     last_setpoint.acceleration = acceleration_setpoint;
    |     last_setpoint.jerk = jerk_setpoint;
    |     last_setpoint.thrust = [single(nan); single(nan); single(nan)];
    | 
    |     % update_initial
    |     FlightTask_updateInitialize;
    |     flag_init = Sticks_checkAndSetStickInputs && isfinite(position_(3)) && isfinite(velocity_(3)) && isfinite(yaw_);
    | 
    |     % active
    |     FlightTaskManualAltitude_activate;
    | 
    |     trajectory.state_j = single(0);
    |     trajectory.state_a = IsFinite(last_setpoint.acceleration(3), single(0));
    |     trajectory.state_v = IsFinite(last_setpoint.vz, velocity_(3));
    |     trajectory.state_x = IsFinite(last_setpoint.z, position_(3));
    |     trajectory.state_init_j = trajectory.state_j;
    |     trajectory.state_init_a = trajectory.state_a;
    |     trajectory.state_init_v = trajectory.state_v;
    |     trajectory.state_init_x = trajectory.state_x;
    | 
    |     position_lock_active_z = false;
    |     position_setpoint_locked = single(nan);
    | 
    |     out = flag_init;
    |     % out = true;
    | end
    | 
    | end
  function Failsafe_update:
    | function Failsafe_update
    | 
    | % checkEkfResetCounters
    | if local_position.xy_reset_counter ~= reset_counter_xy_
    |     reset_counter_xy_ = local_position.xy_reset_counter;
    | end
    | 
    | if local_position.vxy_reset_counter ~= reset_counter_vxy_
    |     reset_counter_vxy_ = local_position.vxy_reset_counter;
    | end
    | 
    | if local_position.z_reset_counter ~= reset_counter_z_
    |     reset_counter_z_ = local_position.z_reset_counter;
    | end
    | 
    | if local_position.vz_reset_counter ~= reset_counter_vz_
    |     reset_counter_vz_ = local_position.vz_reset_counter;
    | end
    | 
    | if local_position.heading_reset_counter ~= reset_counter_heading_
    |     reset_counter_heading_ = local_position.heading_reset_counter;
    | end
    | 
    | % update setpoints
    | if isfinite(position_(1)) && isfinite(position_(2))
    |     velocity_setpoint(1) = single(0);
    |     velocity_setpoint(2) = single(0);
    |     acceleration_setpoint(1) = single(0);
    |     acceleration_setpoint(2) = single(0);
    | elseif isfinite(velocity_(1)) && isfinite(velocity_(2))
    |     position_setpoint(1) = single(nan);
    |     position_setpoint(2) = single(nan);
    |     acceleration_setpoint(1) = single(nan);
    |     acceleration_setpoint(2) = single(nan);
    | end
    | 
    | if isfinite(position_(3))
    |     velocity_setpoint(3) = single(0);
    |     acceleration_setpoint(3) = single(nan);
    | elseif isfinite(velocity_(3))
    |     velocity_setpoint(3) = MPC_LAND_SPEED;
    |     position_setpoint(3) = single(nan);
    |     acceleration_setpoint(3) = single(nan);
    | end
    | 
    | end
  function takeoff_reactivate:
    | function takeoff_reactivate
    | 
    | if takeoff_state < uint8(PX4_TAKEOFF_STATUS.TAKEOFF_STATE_RAMPUP)
    |     FlightTask_activate;
    | end
    | 
    | end
  function out = switchTask:
    | function out = switchTask
    | out = true;
    | 
    | if task_ ~= task_last_
    |     FlightTask_updateInitialize;
    |     FlightTask_activate;
    |     
    |     position_setpoint = position_;
    |     velocity_setpoint = [single(0); single(0); single(0)];
    |     acceleration_setpoint = [single(0); single(0); single(0.3)];
    |     yaw_setpoint = yaw_;
    |     yawspeed_setpoint = single(0);
    | end
    | 
    | end
  function FlightTask_updateInitialize:
    | function FlightTask_updateInitialize()
    | 
    | % 超时时间：0.5s
    | timeout = 0.5;
    | deltatime_ = min((getSimulationTime - time_stamp_last_), timeout);
    | time_stamp_last_ = getSimulationTime;
    | 
    | % evaluateVehicleLocalPosition()
    | position_ = single([nan; nan; nan]);
    | velocity_ = single([nan; nan; nan]);
    | yaw_ = single(nan);
    | dist_to_bottom_ = single(nan);
    | 
    | % 如果local_position这个topic距离当前的时间不超过0.5s，该主题内容有效
    | if ((getSimulationTime - local_position.timestamp) < timeout)
    |     
    |     % 航向
    |     yaw_ = local_position.heading;
    |     
    |     % 水平位置
    |     if (local_position.xy_valid)
    |         position_(1) = local_position.x;
    |         position_(2) = local_position.y;
    |     end
    |     
    |     % 垂直位置
    |     if (local_position.z_valid)
    |         position_(3) = local_position.z;
    |     end
    |     
    |     % 水平速度
    |     if (local_position.v_xy_valid)
    |         velocity_(1) = local_position.vx;
    |         velocity_(2) = local_position.vy;
    |     end
    |     
    |     % 垂直速度
    |     if (local_position.v_z_valid)
    |         velocity_(3) = local_position.vz;
    |     end
    |     
    |     % 对地高度
    |     if (local_position.dist_bottom_valid && isfinite(local_position.dist_bottom))
    |         dist_to_bottom_ = local_position.dist_bottom;
    |     end
    |     
    | end
    | 
    | % evaluateVehicleLocalPositionSetpoint()
    | % only used in Manual Mode
    | if (hasChanged(position_setpoint_input.timestamp) && (getSimulationTime - position_setpoint_input.timestamp) < timeout)
    |     velocity_setpoint_feedback_ = [position_setpoint_input.vx; position_setpoint_input.vy; position_setpoint_input.vz];
    |     acceleration_setpoint_feedback = position_setpoint_input.acceleration;
    | else
    |     velocity_setpoint_feedback_ = single([nan; nan; nan]);
    |     acceleration_setpoint_feedback = single([nan; nan; nan]);
    | end
    | 
    | % evaluateDistanceToGround()
    | if (isfinite(dist_to_bottom_))
    |     dist_to_ground_ = dist_to_bottom_;
    | elseif (home_position.valid_alt)
    |     dist_to_ground_ = -(position_(3) - home_position.z);
    | else
    |     dist_to_ground_ = -position_(3);
    | end
    | 
    | end
  function FlightTask_activate:
    | function FlightTask_activate()
    | 
    | % _resetSetpoints()
    | position_setpoint     = single([nan; nan; nan]);
    | velocity_setpoint     = single([nan; nan; nan]);
    | acceleration_setpoint = single([nan; nan; nan]);
    | jerk_setpoint         = single([nan; nan; nan]);
    | yaw_setpoint          = single(nan);
    | yawspeed_setpoint     = single(nan);
    | 
    | % _setDefaultConstraints()
    | constraints = setDefaultConstraint();
    | 
    | end
    | 
    | function y = setDefaultConstraint()
    | 
    | y.timestamp    = uint64(getSimulationTime * 1e+6);
    | y.speed_xy     = single(MPC_XY_VEL_MAX);
    | y.speed_up     = single(MPC_Z_VEL_MAX_UP);
    | y.speed_down   = single(MPC_Z_VEL_MAX_DN);
    | y.want_takeoff = false;
    |  
    | end
  function FlightTaskManualAltitude_activate:
    | function FlightTaskManualAltitude_activate()
    | 
    | mode_action.FlightTask_activate();
    | 
    | yaw_setpoint = single(nan);
    | yawspeed_setpoint = single(0.0);
    | acceleration_setpoint = single([0.0; 0.0; nan]);
    | position_setpoint(3) = position_(3);
    | velocity_setpoint(3) = single(0.0);
    | 
    | mode_action.FlightTaskManualAltitude_updateConstraintsFromEstimator();
    | 
    | max_speed_up_   = constraints.speed_up;
    | max_speed_down_ = constraints.speed_down;
    | 
    | end
  function FlightTaskManualAltitude_updateConstraintsFromEstimator:
    | function FlightTaskManualAltitude_updateConstraintsFromEstimator()
    | 
    | if (isfinite(local_position.hagl_min))
    |     min_distance_to_ground_ = local_position.hagl_min;
    | else
    |     min_distance_to_ground_ = -single(inf);
    | end
    | 
    | if (isfinite(local_position.hagl_max))
    |     max_distance_to_ground_ = local_position.hagl_max;
    | else
    |     max_distance_to_ground_ = single(inf);
    | end
    | 
    | end
  function input_available = Sticks_checkAndSetStickInputs:
    | function input_available = Sticks_checkAndSetStickInputs()
    | 
    | input_available = true;
    | 
    | if (hasChanged(manual_control_setpoint.timestamp))
    |     % 线性缩放
    |     stick_positions_(1) = manual_control_setpoint.x;    % NED x, pitch [-1,1]
    |     stick_positions_(2) = manual_control_setpoint.y;    % NED y, roll [-1,1]
    |     stick_positions_(3) = (constrain(manual_control_setpoint.z, single(0.0), single(1.0)) - 0.5) * 2;    % NED z, thrust resacaled from [0,1] to [-1,1]
    |     stick_positions_(4) = manual_control_setpoint.r;    % yaw [-1,1]
    |     
    |     % 指数缩放
    |     positions_expo_(1) = expo_deadzone(stick_positions_(1), MPC_XY_MAN_EXPO, MPC_HOLD_DZ);
    |     positions_expo_(2) = expo_deadzone(stick_positions_(2), MPC_XY_MAN_EXPO, MPC_HOLD_DZ);
    |     positions_expo_(3) = expo_deadzone(stick_positions_(3), MPC_Z_MAN_EXPO, MPC_HOLD_DZ);
    |     positions_expo_(4) = expo_deadzone(stick_positions_(4), MPC_YAW_EXPO, MPC_HOLD_DZ);
    |     
    |     % 检查杆量是否有效
    |     input_available = isfinite(stick_positions_(1)) && isfinite(stick_positions_(2)) && isfinite(stick_positions_(3)) && isfinite(stick_positions_(4));
    | else
    |     if ((hasChanged(vehicle_status.timestamp)) && (vehicle_status.rc_signal_lost))
    |         input_available = false;
    |     end
    | end
    | 
    | if (~input_available)
    |     stick_positions_ = single(zeros(4, 1));
    |     positions_expo_  = single(zeros(4, 1));
    | end
    | 
    | input_available = input_available;
    | 
    | end
  function out = VelocitySmoothing_updateTraj(dt,time_stretch,traj):
    | function out = VelocitySmoothing_updateTraj(dt,time_stretch,traj)
    | 
    | out = traj;
    | 
    | out.local_time = traj.local_time + dt * time_stretch;
    | t_remain = out.local_time;
    | 
    | t1 = min(t_remain, traj.T1);
    | [state_j, state_a, state_v, state_x] = evaluatePoly(traj.max_jerk, traj.state_init_a, traj.state_init_v, traj.state_init_x, t1, traj.direction);
    | t_remain = t_remain - t1;
    | 
    | if t_remain > single(0)
    |     t2 = min(t_remain, traj.T2);
    |     [state_j, state_a, state_v, state_x] = evaluatePoly(single(0), state_a, state_v, state_x, t2, single(0));
    |     t_remain = t_remain - t2;
    | end
    | 
    | if t_remain > single(0)
    |     t3 = min(t_remain, traj.T3);
    |     [state_j, state_a, state_v, state_x] = evaluatePoly(traj.max_jerk, state_a, state_v, state_x, t3, -traj.direction);
    |     t_remain = t_remain - t3;
    | end
    | 
    | if t_remain > single(0)
    |     [state_j, state_a, state_v, state_x] = evaluatePoly(single(0), single(0), state_v, state_x, t_remain, single(0));
    | end
    | 
    | out.state_j = state_j;
    | out.state_a = state_a;
    | out.state_v = state_v;
    | out.state_x = state_x;
    | 
    | end
  function out = VelocitySmoothing_updateDurations(vel_setpoint,traj):
    | function out = VelocitySmoothing_updateDurations(vel_setpoint,traj)
    | out = traj;
    | 
    | out.vel_sp = constrain(vel_setpoint, -traj.max_vel, traj.max_vel);
    | out.local_time = single(0);
    | out.state_init_x = traj.state_x;
    | out.state_init_v = traj.state_v;
    | out.state_init_a = traj.state_a;
    | out.state_init_j = traj.state_j;
    | 
    | out.direction = int32(computeDirection(traj.state_v,traj.state_a,traj.max_jerk,out.vel_sp));
    | 
    | if out.direction ~= 0
    |     [out.T1, out.T2, out.T3] = updateDurationsMinimizeTotalTime(out.direction,traj.max_jerk,traj.max_accel,out.vel_sp,traj.state_a,traj.state_v);
    | else
    |     out.T1 = single(0);
    |     out.T2 = single(0);
    |     out.T3 = single(0);
    | end
    | 
    | end
    | 
    | %% 
    | function y = computeDirection(state_v,state_a,max_jerk,velsp)
    | 
    | vel_zero_acc = computeVelAtZeroAcc(state_v,state_a,max_jerk);
    | 
    | y = sign(velsp - vel_zero_acc);
    | 
    | if y == 0
    |     y = sign(state_a);
    | end
    | 
    | end
    | 
    | %% 
    | function y = computeVelAtZeroAcc(state_v,state_a,max_jerk)
    | 
    | y = state_v;
    | 
    | if abs(state_a) > eps
    |     j_zero_acc = -sign(state_a) * max_jerk;
    |     t_zero_acc = -state_a / j_zero_acc;
    |     y = state_v + state_a * t_zero_acc + 0.5 * j_zero_acc * t_zero_acc * t_zero_acc;
    | end
    | 
    | end
    | 
    | %% 
    | function [t1,t2,t3] = updateDurationsMinimizeTotalTime(dir,max_jerk,max_accel,velsp,state_a,state_v)
    | 
    | jerk_max_T1 = single(dir) * max_jerk;
    | delta_v = velsp - state_v;
    | 
    | t1 = computeT1(state_a, delta_v, jerk_max_T1, max_accel);
    | t3 = computeT3(t1, state_a, jerk_max_T1);
    | t2 = computeT2(t1, t3, state_a, delta_v, jerk_max_T1);
    | 
    | end
    | 
    | %% 
    | function y = computeT1(a0, v3, j_max, a_max)
    | 
    | delta = 2 * a0 * a0 + 4 * j_max * v3;
    | 
    | if delta < 0
    |     y = single(0);
    | else
    |     sqrt_delta = sqrt(delta);
    |     T1_plus = (-a0 + 0.5 * sqrt_delta) / j_max;
    |     T1_minus = (-a0 - 0.5 * sqrt_delta) / j_max;
    |     
    |     T3_plus = a0 / j_max + T1_plus;
    |     T3_minus = a0 / j_max + T1_minus;
    |     
    |     if (T1_plus >= single(0)) && (T3_plus >= single(0))
    |         t1 = T1_plus;
    |     elseif (T1_minus >= single(0)) && (T3_minus >= single(0))
    |         t1 = T1_minus;
    |     else
    |         t1 = single(0);
    |     end
    |     
    |     t1 = saturateT1ForAccel(a0, j_max, t1, a_max);
    |     y = max(t1, single(0));
    | end
    | 
    | end
    | 
    | %% 
    | function y = computeT2(t1, t3, a0, v3, j_max)
    | 
    | den = a0 + j_max * t1;
    | if den <= single(0)
    |     den = -den;
    | end
    | 
    | if den > eps
    |     t2 = (-0.5 * t1^2 * j_max - t1 * t3 * j_max - t1 * a0 + 0.5 * t3^2 * j_max - t3 * a0 + v3) / den;
    | else
    |     t2 = single(0);
    | end
    | 
    | y = max(t2, single(0));
    | 
    | end
    | 
    | %% 
    | function y = computeT3(t1, a0, j_max)
    | 
    | t3 = a0 / j_max + t1;
    | y = max(t3, single(0));
    | 
    | end
    | 
    | %% 
    | function y = saturateT1ForAccel(a0, j_max, t1, a_max)
    | 
    | accel_T1 = a0 + j_max * t1;
    | 
    | if accel_T1 > a_max
    |     y = (a_max - a0) / j_max;
    | elseif accel_T1 < -a_max
    |     y = (-a_max - a0) / j_max;
    | else
    |     y = t1;
    | end
    | 
    | end
  function out = VelocitySmoothing_timeSynchronization(traj, n_traj):
    | function out = VelocitySmoothing_timeSynchronization(traj, n_traj)
    | 
    | out = traj;
    | 
    | desired_time = single(0);
    | longest_traj_index = single(0);
    | 
    | for i = 1:1:n_traj
    |     T123 = traj(i).T1 + traj(i).T2 + traj(i).T3;
    |     
    |     if T123 > desired_time
    |         desired_time = T123;
    |         longest_traj_index = single(i);
    |     end
    | end
    | 
    | if desired_time > eps
    |     for i = 1:1:n_traj
    |         if i ~= longest_traj_index
    |             out(i) = updateDurationsGivenTotalTime(desired_time, traj(i));
    |         end
    |     end
    | end
    | 
    | end
    | 
    | %% 
    | function oout = updateDurationsGivenTotalTime(T123,ttraj)
    | oout = ttraj;
    | 
    | jerk_max_T1 = single(ttraj.direction) * ttraj.max_jerk;
    | delta_v = ttraj.vel_sp - ttraj.state_v;
    | 
    | oout.T1 = computeT11(T123, ttraj.state_a, delta_v, jerk_max_T1, ttraj.max_accel);
    | oout.T3 = computeT33(oout.T1, ttraj.state_a, jerk_max_T1);
    | oout.T2 = computeT22(T123, oout.T1, oout.T3);
    | 
    | end
    | 
    | %% 
    | function y = computeT11(T123, a0, v3, j_max, a_max)
    | 
    | a = -j_max;
    | b = j_max * T123 - a0;
    | delta = T123^2 * j_max^2 + 2 * T123 * a0 * j_max - a0^2 - 4 * j_max * v3;
    | 
    | if delta < 0
    |     y = single(0);
    | else
    |     sqrt_delta = sqrt(delta);
    |     denominator_inv = 1 / (2 * a);
    |     T1_plus = max((-b + sqrt_delta) * denominator_inv, single(0));
    |     T1_minus = max((-b - sqrt_delta) * denominator_inv, single(0));
    |     
    |     T3_plus = a0 / j_max + T1_plus;
    |     T3_minus = a0 / j_max + T1_minus;
    |     
    |     T13_plus = T1_plus + T3_plus;
    |     T13_minus = T1_minus + T3_minus;
    |     
    |     if T13_plus > T123
    |         t1 = T1_minus;
    |     elseif T13_minus > T123
    |         t1 = T1_plus;
    |     else
    |         t1 = single(0);
    |     end
    |     
    |     y = saturateT1ForAccel(a0, j_max, t1, a_max);
    | end
    | 
    | end
    | 
    | %% 
    | function y = computeT22(T123, t1, t3)
    | 
    | t2 = T123 - t1 - t3;
    | y = max(t2, single(0));
    | 
    | end
    | 
    | %% 
    | function y = computeT33(t1, a0, j_max)
    | 
    | t3 = a0 / j_max + t1;
    | y = max(t3, single(0));
    | 
    | end
    | 
    | %% 
    | function y = saturateT1ForAccel(a0, j_max, t1, a_max)
    | 
    | accel_T1 = a0 + j_max * t1;
    | 
    | if accel_T1 > a_max
    |     y = (a_max - a0) / j_max;
    | elseif accel_T1 < -a_max
    |     y = (-a_max - a0) / j_max;
    | else
    |     y = single(t1);
    | end
    | 
    | end
  function out = rotateIntoHeadingFrame(u):
    | function out = rotateIntoHeadingFrame(u)
    | 
    | yaw_rotate = IsFinite(yaw_setpoint, yaw_);
    | v_r = Euler2DCM(single(0), single(0), yaw_rotate) * [u(1); u(2); single(0)];
    | 
    | out = [v_r(1), v_r(2)];
    | 
    | end
  function respectMaxAltitude:
    | function respectMaxAltitude
    | 
    | if isfinite(dist_to_bottom_)
    |     if isfinite(max_distance_to_ground_)
    |         constraints.speed_up = constrain(MPC_Z_P * (max_distance_to_ground_ - dist_to_bottom_), -max_speed_down_, max_speed_up_);
    |     else
    |         constraints.speed_up = max_speed_up_;
    |     end
    |     
    |     if dist_to_bottom_ > max_distance_to_ground_
    |         position_setpoint(3) = position_(3) + (dist_to_bottom_ - max_distance_to_ground_);
    |         constraints.speed_down = min(max_speed_down_, 0.7);
    |     else
    |         constraints.speed_down = max_speed_down_;
    |     end
    | end
    | 
    | end
  function out = terrainFollowing(apply_brake, stopped, d_to_g_lock):
    | function out = terrainFollowing(apply_brake, stopped, d_to_g_lock)
    | 
    | if apply_brake && stopped && ~isfinite(d_to_g_lock)
    |     position_setpoint(3) = position_(3);
    |     if isfinite(dist_to_bottom_) && (dist_to_bottom_ < min_distance_to_ground_)
    |         position_setpoint(3) = position_(3) - (min_distance_to_ground_ - dist_to_bottom_);
    |     end
    |     out = dist_to_bottom_ - (position_setpoint(3) - position_(3));
    |     
    | elseif apply_brake && isfinite(d_to_g_lock)
    |     position_setpoint(3) = position_(3) - (d_to_g_lock - dist_to_bottom_);
    |     out = d_to_g_lock;
    |     
    | else
    |     position_setpoint(3) = single(nan);
    |     out = single(nan);    
    | end
    | 
    | end
  function out = get_weathervane_yawrate(dcm_z, yyaw):
    | function out = get_weathervane_yawrate(dcm_z, yyaw)
    | 
    | body_z_sp = dcm_z;
    | R_yaw = Euler2DCM(0, 0, yyaw);
    | body_z_sp = R_yaw * body_z_sp;
    | body_z_sp = body_z_sp / norm(body_z_sp);
    | 
    | roll_sp = -asin(body_z_sp(2));
    | min_roll_rad = deg2rad(WV_ROLL_MIN);
    | 
    | if roll_sp > min_roll_rad
    |     roll_exceeding_treshold = roll_sp - min_roll_rad;
    | elseif roll_sp < -min_roll_rad
    |     roll_exceeding_treshold = roll_sp + min_roll_rad;
    | else
    |     roll_exceeding_treshold = single(0);
    | end
    | 
    | out = constrain(roll_exceeding_treshold * WV_GAIN, -deg2rad(WV_YRATE_MAX), deg2rad(WV_YRATE_MAX));
    | 
    | end
